simulink library "outp"  (R2021b)
settings: Solver=VariableStepAuto  StartTime=0.0  StopTime=10.0  RelTol=1e-3
undefined symbols (not defined in the file or in its folder): ENUM_PMMMODE_CHARGE, ENUM_PMMMODE_IDLE, ENUM_PMMMODE_INITIALIZE, ENUM_PMMMODE_POWERDOWN, ENUM_PMMMODE_SLEEP, Left, outp, slcm, TRUE
libraries: FVT_lib x686, hcu_lib x4, simulink x1
(part 4 of 7)

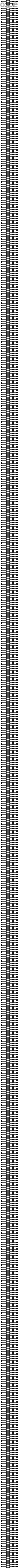
== system outp/OUTP/outpmodule ==
  VACC_HVTHCMSysAvail_enum : Inport
  VACC_LVBattVoltSta_enum : Inport  Port=2
  VACC_VehHVPwrAvail4THCM_W : Inport  Port=3
  VAPM_VehSpeed_kph : Inport  Port=4
  VAPM_VehSpeedTimeOut_flg : Inport  Port=5
  VAPM_FSOffSw_enum : Inport  Port=6
  VAPM_FSOffSwTimeOut_flg : Inport  Port=7
  VAPM_ChrgPlugSta_enum : Inport  Port=8
  VAPM_PASDRMR_cm : Inport  Port=9
  VAPM_PASDRML_cm : Inport  Port=10
  VAPM_PASDRCR_cm : Inport  Port=11
  VAPM_PASDRCL_cm : Inport  Port=12
  VAPM_PASDFMR_cm : Inport  Port=13
  VAPM_PASDFML_cm : Inport  Port=14
  VAPM_PASDFCR_cm : Inport  Port=15
  VAPM_PASDFCL_cm : Inport  Port=16
  VAPM_APSDRLR_cm : Inport  Port=17
  VAPM_APSDRLL_cm : Inport  Port=18
  VAPM_APSDFLR_cm : Inport  Port=19
  VAPM_APSDFLL_cm : Inport  Port=20
  VAPM_PASAFCL_enum : Inport  Port=21
  VAPM_PASARMR_enum : Inport  Port=22
  VAPM_PASARML_enum : Inport  Port=23
  VAPM_PASARCR_enum : Inport  Port=24
  VAPM_PASARCL_enum : Inport  Port=25
  VAPM_PASAFMR_enum : Inport  Port=26
  VAPM_PASAFML_enum : Inport  Port=27
  VAPM_PASAFCR_enum : Inport  Port=28
  VAPM_USSStaRMR_flg : Inport  Port=29
  VAPM_USSStaRML_flg : Inport  Port=30
  VAPM_USSStaRLR_flg : Inport  Port=31
  VAPM_USSStaRLL_flg : Inport  Port=32
  VAPM_USSStaRCR_flg : Inport  Port=33
  VAPM_USSStaRCL_flg : Inport  Port=34
  VAPM_USSStaFMR_flg : Inport  Port=35
  VAPM_USSStaFML_flg : Inport  Port=36
  VAPM_USSStaFLR_flg : Inport  Port=37
  VAPM_USSStaFLL_flg : Inport  Port=38
  VAPM_USSStaFCR_flg : Inport  Port=39
  VAPM_USSStaFCL_flg : Inport  Port=40
  VAPM_Chime_enum : Inport  Port=41
  VAPM_SNSRLayout_enum : Inport  Port=42
  VAPM_StaFSya_flg : Inport  Port=43
  VAPM_ModOperation_enum : Inport  Port=44
  VAPM_BrkPedalPos_pct : Inport  Port=45
  VAPM_BrkPedalPosTimeOut_flg : Inport  Port=46
  VAPM_LFRawWhlSpeed_kph : Inport  Port=47
  VAPM_LFRawWhlSpeedTimeOut_flg : Inport  Port=48
  VAPM_RFRawWhlSpeed_kph : Inport  Port=49
  VAPM_RFRawWhlSpeedTimeOut_flg : Inport  Port=50
  VAPM_LRRawWhlSpeed_kph : Inport  Port=51
  VAPM_LRRawWhlSpeedTimeOut_flg : Inport  Port=52
  VAPM_RRRawWhlSpeed_kph : Inport  Port=53
  VAPM_RRRawWhlSpeedTimeOut_flg : Inport  Port=54
  VAPM_LFRawWhlSpeedV_flg : Inport  Port=55
  VAPM_LFRawWhlSpeedVTimeOut_flg : Inport  Port=56
  VAPM_RFRawWhlSpeedV_flg : Inport  Port=57
  VAPM_RFRawWhlSpeedVTimeOut_flg : Inport  Port=58
  VAPM_LRRawWhlSpeedV_flg : Inport  Port=59
  VAPM_LRRawWhlSpeedVTimeOut_flg : Inport  Port=60
  VAPM_RRRawWhlSpeedV_flg : Inport  Port=61
  VAPM_RRRawWhlSpeedVTimeOut_flg : Inport  Port=62
  VAPM_LFWhlRotDir_enum : Inport  Port=63
  VAPM_LFWhlRotDirTimeOut_flg : Inport  Port=64
  VAPM_RFWhlRotDir_enum : Inport  Port=65
  VAPM_RFWhlRotDirTimeOut_flg : Inport  Port=66
  VAPM_LRWhlRotDir_enum : Inport  Port=67
  VAPM_LRWhlRotDirTimeOut_flg : Inport  Port=68
  VAPM_RRWhlRotDir_enum : Inport  Port=69
  VAPM_RRWhlRotDirTimeOut_flg : Inport  Port=70
  VAPM_LFPulseCountV_flg : Inport  Port=71
  VAPM_LFPulseCountVTimeOut_flg : Inport  Port=72
  VAPM_RFPulseCountV_flg : Inport  Port=73
  VAPM_RFPulseCountVTimeOut_flg : Inport  Port=74
  VAPM_LRPulseCountV_flg : Inport  Port=75
  VAPM_LRPulseCountVTimeOut_flg : Inport  Port=76
  VAPM_RRPulseCountV_flg : Inport  Port=77
  VAPM_RRPulseCountVTimeOut_flg : Inport  Port=78
  VAPM_LFPulseCount_enum : Inport  Port=79
  VAPM_LFPulseCountTimeOut_flg : Inport  Port=80
  VAPM_RFPulseCount_enum : Inport  Port=81
  VAPM_RFPulseCountTimeOut_flg : Inport  Port=82
  VAPM_LRPulseCount_enum : Inport  Port=83
  VAPM_LRPulseCountTimeOut_flg : Inport  Port=84
  VAPM_RRPulseCount_enum : Inport  Port=85
  VAPM_RRPulseCountTimeOut_flg : Inport  Port=86
  VAPM_ShifterHandleCmd_enum : Inport  Port=87
  VAPM_ShifterHandleCmdTimeOut_flg : Inport  Port=88
  VAPM_DriIntend_enum : Inport  Port=89
  VAPM_DriIntendTimeOut_flg : Inport  Port=90
  VAPM_EPSAOIControl_enum : Inport  Port=91
  VAPM_EPSAOIControlTimeOut_flg : Inport  Port=92
  VAPM_SASAngle_Deg : Inport  Port=93
  VAPM_SASAngleTimeOut_flg : Inport  Port=94
  VAPM_SASSpeed_degps : Inport  Port=95
  VAPM_SASSpeedTimeOut_flg : Inport  Port=96
  VAPM_SASSpeedValid_flg : Inport  Port=97
  VAPM_SASSpeedValidTimeOut_flg : Inport  Port=98
  VAPM_SASCAL_flg : Inport  Port=99
  VAPM_SASCALTimeOut_flg : Inport  Port=100
  VAPM_SASV_flg : Inport  Port=101
  VAPM_SASVTimeOut_flg : Inport  Port=102
  VAPM_GRADE_Deg : Inport  Port=103
  VAPM_GRADETimeOut_flg : Inport  Port=104
  VAPM_YawRate_degps : Inport  Port=105
  VAPM_YawRateTimeOut_flg : Inport  Port=106
  VAPM_LatAccel_Gps : Inport  Port=107
  VAPM_LatAccelTimeOut_flg : Inport  Port=108
  VAPM_LongAccel_Gps : Inport  Port=109
  VAPM_LongAccelTimeOut_flg : Inport  Port=110
  VAPM_MCPressure_bar : Inport  Port=111
  VAPM_MCPressureTimeOut_flg : Inport  Port=112
  VAPM_YawRateV_flg : Inport  Port=113
  VAPM_YawRateVTimeOut_flg : Inport  Port=114
  VAPM_LatAccelV_flg : Inport  Port=115
  VAPM_LatAccelVTimeOut_flg : Inport  Port=116
  VAPM_LongAccelV_flg : Inport  Port=117
  VAPM_LongAccelVTimeOut_flg : Inport  Port=118
  VAPM_MCPressureV_bar : Inport  Port=119
  VAPM_MCPressureVTimeOut_flg : Inport  Port=120
  VAPM_BrkSwSta_flg : Inport  Port=121
  VAPM_BrkSwStaTimeOut_flg : Inport  Port=122
  VAPM_BrkSwV_flg : Inport  Port=123
  VAPM_BrkSwVTimeOut_flg : Inport  Port=124
  VAPM_ESCStandstill_flg : Inport  Port=125
  VAPM_ESCStandstillTimeOut_flg : Inport  Port=126
  VAPM_ESCAPSSta_enum : Inport  Port=127
  VAPM_ESCAPSStaTimeOut_flg : Inport  Port=128
  VAPM_EPBExtReleaseAvail_flg : Inport  Port=129
  VAPM_EPBExtReleaseAvailTimeOut_flg : Inport  Port=130
  VAPM_EPBExtApplyAvail_flg : Inport  Port=131
  VAPM_EPBExtApplyAvailTimeOut_flg : Inport  Port=132
  VAPM_EPBErrSta_enum : Inport  Port=133
  VAPM_EPBErrStaTimeOut_flg : Inport  Port=134
  VAPM_EPBSta_enum : Inport  Port=135
  VAPM_EPBStaTimeOut_flg : Inport  Port=136
  VAPM_AVMparkingcancel_enum : Inport  Port=137
  VAPM_AVMparkingcancelTimeOut_flg : Inport  Port=138
  VAPM_AVMparkingexcute_enum : Inport  Port=139
  VAPM_AVMparkingexcuteTimeOut_flg : Inport  Port=140
  VAPM_AVMParkingmode_enum : Inport  Port=141
  VAPM_AVMParkingmodeTimeOut_flg : Inport  Port=142
  VAPM_AVMErrSTA_flg : Inport  Port=143
  VAPM_AVMErrSTATimeOut_flg : Inport  Port=144
  VAPM_IVIStatus_flg : Inport  Port=145
  VAPM_IVIStatusTimeOut_flg : Inport  Port=146
  VAPM_CAASSw_enum : Inport  Port=147
  VAPM_CAASSwTimeOut_flg : Inport  Port=148
  VAPM_IVIScreen_enum : Inport  Port=149
  VAPM_IVIScreenTimeOut_flg : Inport  Port=150
  VAPM_ABSActive_flg : Inport  Port=151
  VAPM_ABSActiveTimeOut_flg : Inport  Port=152
  VAPM_TCSActive_flg : Inport  Port=153
  VAPM_TCSActiveTimeOut_flg : Inport  Port=154
  VAPM_DriverSeatBeltCmd_flg : Inport  Port=155
  VAPM_DriverSeatBeltCmdTimeOut_flg : Inport  Port=156
  VAPM_APSProgressPCT_pct : Inport  Port=157
  VAPM_APSRQDisplay_enum : Inport  Port=158
  VAPM_APSSWVer_enum : Inport  Port=159
  VAPM_APSHWVer_enum : Inport  Port=160
  VAPM_APSExitCondition_enum : Inport  Port=161
  VAPM_APSAngleTarget_Deg : Inport  Port=162
  VAPM_APSVRqEPASCtrl_flg : Inport  Port=163
  VAPM_APSRqEPASCtrl_flg : Inport  Port=164
  VAPM_CAASSta_enum : Inport  Port=165
  VBCM_AntitheftSta_enum : Inport  Port=166
  VBCM_TailgateRemote_enum : Inport  Port=167
  VBCM_HornCtrl_flg : Inport  Port=168
  VBCM_AllDoorSW_flg : Inport  Port=169
  VBCM_BCMDoorLockSta_flg : Inport  Port=170
  VBCM_AntitheftSeatFlod_flg : Inport  Port=171
  VBCM_HoodSW_flg : Inport  Port=172
  VBCM_TailgateSW_flg : Inport  Port=173
  VBCM_DrDoorSW_flg : Inport  Port=174
  VBCM_PsDoorSW_flg : Inport  Port=175
  VBCM_RLDoorSW_flg : Inport  Port=176
  VBCM_RRDoorSW_flg : Inport  Port=177
  VBCM_LockSetting_flg : Inport  Port=178
  VBCM_FrChargingDoorCtrl_enum : Inport  Port=179
  VBCM_RrChargingDoorCtrl_enum : Inport  Port=180
  VBCM_CrashDetd_flg : Inport  Port=181
  VBCM_CTDCtrl_enum : Inport  Port=182
  VBCM_DoorLockIND_flg : Inport  Port=183
  VBCM_CTDLockSW_flg : Inport  Port=184
  VBCM_Dimmer_pct : Inport  Port=185
  VBCM_DimmerEN_flg : Inport  Port=186
  VBCM_PosLamp_flg : Inport  Port=187
  VBCM_LBeam_flg : Inport  Port=188
  VBCM_HBeam_flg : Inport  Port=189
  VBCM_RrFogLamp_flg : Inport  Port=190
  VBCM_BrakeLamp_flg : Inport  Port=191
  VBCM_ReverseLamp_flg : Inport  Port=192
  VBCM_LDRL_flg : Inport  Port=193
  VBCM_RDRL_flg : Inport  Port=194
  VBCM_LBSD_flg : Inport  Port=195
  VBCM_RBSD_flg : Inport  Port=196
  VBCM_HazardSW_flg : Inport  Port=197
  VBCM_LTurnLP_flg : Inport  Port=198
  VBCM_RTurnLP_flg : Inport  Port=199
  VBCM_BCMBuzzerReq_flg : Inport  Port=200
  VBCM_MirrorCtrl_enum : Inport  Port=201
  VBCM_MirrorDefog_flg : Inport  Port=202
  VBCM_RrDefog_flg : Inport  Port=203
  VBCM_RoomLampH_flg : Inport  Port=204
  VBCM_RoomLampL_flg : Inport  Port=205
  VBCM_TrunkRel_flg : Inport  Port=206
  VBCM_TailgateHDSW_flg : Inport  Port=207
  VBCM_FrWiperL_flg : Inport  Port=208
  VBCM_FrWiperH_flg : Inport  Port=209
  VBCM_RrWiper_flg : Inport  Port=210
  VBCM_WasherCtrl_enum : Inport  Port=211
  VBCM_WiperFixMode_flg : Inport  Port=212
  VBCM_AmbLightBreath1_enum : Inport  Port=213
  VBCM_AmbLightBreath2_enum : Inport  Port=214
  VBCM_AmbLightBreath3_enum : Inport  Port=215
  VBCM_AmbLightBreath4_enum : Inport  Port=216
  VBCM_AmbLightBreath5_enum : Inport  Port=217
  VBCM_AmbLightBreath6_enum : Inport  Port=218
  VBCM_AmbLightBrightness1_enum : Inport  Port=219
  VBCM_AmbLightBrightness2_enum : Inport  Port=220
  VBCM_AmbLightBrightness3_enum : Inport  Port=221
  VBCM_AmbLightBrightness4_enum : Inport  Port=222
  VBCM_AmbLightBrightness5_enum : Inport  Port=223
  VBCM_AmbLightBrightness6_enum : Inport  Port=224
  VBCM_AmbLightColor1_enum : Inport  Port=225
  VBCM_AmbLightColor2_enum : Inport  Port=226
  VBCM_AmbLightColor3_enum : Inport  Port=227
  VBCM_AmbLightColor4_enum : Inport  Port=228
  VBCM_AmbLightColor5_enum : Inport  Port=229
  VBCM_AmbLightColor6_enum : Inport  Port=230
  VBCM_LampPwr_flg : Inport  Port=231
  VBCM_SPTGDet_flg : Inport  Port=232
  VBCM_APSOpenPTG_flg : Inport  Port=233
  VBCM_FollowMe_flg : Inport  Port=234
  VBCM_IVIRST_flg : Inport  Port=235
  VBCM_CountAlarm_enum : Inport  Port=236
  VBCM_MFSWTri_flg : Inport  Port=237
  VBCM_MirrorFlodPos_flg : Inport  Port=238
  VBCM_FuelDoorPos_flg : Inport  Port=239
  VBCM_MFRDNBrightReq_pct : Inport  Port=240
  VBCM_RoomLampMode_flg : Inport  Port=241
  VBCM_IVIPTGUSStaSW_flg : Inport  Port=242
  VBCM_PTGInnerSW2_enum : Inport  Port=243
  VBCM_LDrvCtrlCmd_pct : Inport  Port=244
  VBCM_LPasCtrlCmd_pct : Inport  Port=245
  VBCM_LRLDCtrlCmd_pct : Inport  Port=246
  VBCM_LRRDCtrlCmd_pct : Inport  Port=247
  VBCM_APMDoorControlSta_flg : Inport  Port=248
  VBCM_AmbFunEN_flg : Inport  Port=249
  VBCM_AmbWelEN_flg : Inport  Port=250
  VBCM_AmbDimEN_flg : Inport  Port=251
  VBCM_AmbLinkDriSta_flg : Inport  Port=252
  VBCM_AmbPwrWarnEN_flg : Inport  Port=253
  VBCM_AmbODAEN_flg : Inport  Port=254
  VBCM_AmbColorSta_enum : Inport  Port=255
  VBCM_AmbBrightSta_enum : Inport  Port=256
  VBCM_LockAlarm_enum : Inport  Port=257
  VBCM_ATCtrl_enum : Inport  Port=258
  VBCM_fUnlockSingle_flg : Inport  Port=259
  VBCM_UserNow_enum : Inport  Port=260
  VBCM_AmbFunENFlash_enum : Inport  Port=261
  VBCM_AmbWelENFlash_enum : Inport  Port=262
  VBCM_AmbDimENFlash_enum : Inport  Port=263
  VBCM_AmbLinkDriStaFlash_enum : Inport  Port=264
  VBCM_AmbPwrWarnENFlash_enum : Inport  Port=265
  VBCM_AmbODAENFlash_enum : Inport  Port=266
  VBCM_AmbColorSta1_enum : Inport  Port=267
  VBCM_AmbColorSta2_enum : Inport  Port=268
  VBCM_AmbColorSta3_enum : Inport  Port=269
  VBCM_AmbColorSta4_enum : Inport  Port=270
  VBCM_AmbColorSta5_enum : Inport  Port=271
  VBCM_AmbColorSta7_enum : Inport  Port=272
  VBCM_AmbBrightnessSta1_enum : Inport  Port=273
  VBCM_AmbBrightnessSta2_enum : Inport  Port=274
  VBCM_AmbBrightnessSta3_enum : Inport  Port=275
  VBCM_AmbBrightnessSta4_enum : Inport  Port=276
  VBCM_AmbBrightnessSta5_enum : Inport  Port=277
  VBCM_AmbBrightnessSta7_enum : Inport  Port=278
  VBCM_HazardIND_flg : Inport  Port=279
  VBCM_DimSwSta_flg : Inport  Port=280
  VBCM_PassSWSta_flg : Inport  Port=281
  VBCM_FWipSwSta_enum : Inport  Port=282
  VBCM_FWasSwSta_enum : Inport  Port=283
  VBCM_TurnSwSta_enum : Inport  Port=284
  VDHP_ActAPSPosn_pct : Inport  Port=285
  VDHP_EAPS1MIN_pct : Inport  Port=286
  VDHP_EAPS2MIN_pct : Inport  Port=287
  VDKC_DKCTimeSN_cnt : Inport  Port=288
  VDKC_DKCAuthSta_enum : Inport  Port=289
  VDSC_DISCTurn_flg : Inport  Port=290
  VDSC_DISCTargetSpd_kph : Inport  Port=291
  VDSC_DISCSta_enum : Inport  Port=292
  VDSC_DISCButtSta_flg : Inport  Port=293
  VNMM_AllCANTxReq_flg : Inport  Port=294
  VNMM_NMmTxReq_flg : Inport  Port=295
  VNMM_Awake_enum : Inport  Port=296
  VNMM_CSB_flg : Inport  Port=297
  VNMM_ErrorState_enum : Inport  Port=298
  VNMM_NodeID_enum : Inport  Port=299
  VNMM_PNI_flg : Inport  Port=300
  VNMM_RptMsgReq_flg : Inport  Port=301
  VNMM_WakeUp_enum : Inport  Port=302
  VNMM_ActiveWU_flg : Inport  Port=303
  VNMM_SysNMmSta_enum : Inport  Port=304
  VNMM_NetworkReq_flg : Inport  Port=305
  VPMM_PowerUpState_enum : Inport  Port=306
  VPMM_PowerDownState_enum : Inport  Port=307
  VPMM_PowerUpFault_enum : Inport  Port=308
  VPMM_PowerDownFault_enum : Inport  Port=309
  VPMM_ActiveDischargeReq_flg : Inport  Port=310
  VPMM_DCDCEnaReq_flg : Inport  Port=311
  VPMM_DCDCVoltSetpoint_V : Inport  Port=312
  VPMM_HVBatCnctReq_flg : Inport  Port=313
  VPMM_HVSysReadyToCharge_enum : Inport  Port=314
  VPMM_PowerSta_enum : Inport  Port=315
  VPMM_LVPwrSta_flg : Inport  Port=316
  VPMM_HVPwrSta_flg : Inport  Port=317
  VPMM_SysPowerMode_enum : Inport  Port=318
  VPMM_FrMCUEnaReq_flg : Inport  Port=319
  VPMM_RrMCUEnaReq_flg : Inport  Port=320
  VPMM_DrivetrainSelect_enum : Inport  Port=321
  VPMM_DrSeatSta_enum : Inport  Port=322
  VPMM_PwrStaSelect_enum : Inport  Port=323
  VPMM_PwrStaConstraint_enum : Inport  Port=324
  VPMM_TCountSta_enum : Inport  Port=325
  VPMM_PwrUpReq_enum : Inport  Port=326
  VPMM_PwrDownReq_enum : Inport  Port=327
  VPMM_LowSOCWarn_enum : Inport  Port=328
  VPMM_ReVehThdChkSta_enum : Inport  Port=329
  VPMM_LVSysErrPwrOutErr_flg : Inport  Port=330
  VPMM_EvccAplusPwrUpReq_flg : Inport  Port=331
  VPMM_PwrStaONTOPopReq_flg : Inport  Port=332
  VPMM_IVIPwrStaONTOPopT_s : Inport  Port=333
  VPMM_LVChrgHoldTtimer_s : Inport  Port=334
  VPMM_LVBattChrgTimeCnt_s : Inport  Port=335
  VPMM_SilentChkAllowSleep_flg : Inport  Port=336
  VPMM_TimerAllowSleep_flg : Inport  Port=337
  VPMM_FDADC12VDetAvg_mV : Inport  Port=338
  VPMM_PMMAllowECUSleep_flg : Inport  Port=339
  VPMM_LVSilentChrgSta_enum : Inport  Port=340
  VPMM_LVSilentChrgReq_flg : Inport  Port=341
  VPMM_LVSilentChrgLv_enum : Inport  Port=342
  VPMM_CtrlFrPwrStbA1P_flg : Inport  Port=343
  VPMM_CtrlFrRC1_flg : Inport  Port=344
  VPMM_CtrlFrBMSCCUCIR_flg : Inport  Port=345
  VPMM_CtrlFrEDUINVERTER_flg : Inport  Port=346
  VPMM_HWResetSta_enum : Inport  Port=347
  VPMM_CtrlDrPwrStbA2_flg : Inport  Port=348
  VPMM_PwrStaTOSta_enum : Inport  Port=349
  VPMM_Sched_ChgTOSta_enum : Inport  Port=350
  VPMM_PwrReq_OTA_enum : Inport  Port=351
  VPMM_OTAPwrReqOFFChkSta_enum : Inport  Port=352
  VPMM_OTAPwrReqStdChkSta_enum : Inport  Port=353
  VSYS_HWVer1_cnt : Inport  Port=354
  VSYS_HWVer2_cnt : Inport  Port=355
  VSYS_HWVer3_cnt : Inport  Port=356
  VSYS_CarModel1_cnt : Inport  Port=357
  VSYS_CarModel2_cnt : Inport  Port=358
  VSYS_CarModel3_cnt : Inport  Port=359
  VSYS_ECU1_cnt : Inport  Port=360
  VSYS_ECU2_cnt : Inport  Port=361
  VSYS_Major1_cnt : Inport  Port=362
  VSYS_Major2_cnt : Inport  Port=363
  VSYS_Minor1_cnt : Inport  Port=364
  VSYS_Minor2_cnt : Inport  Port=365
  VSYS_Patch1_cnt : Inport  Port=366
  VSYS_Patch2_cnt : Inport  Port=367
  VSYS_Country1_cnt : Inport  Port=368
  VSYS_Country2_cnt : Inport  Port=369
  VSYS_Variation_cnt : Inport  Port=370
  VSYS_Dash1_cnt : Inport  Port=371
  VSYS_Change1_cnt : Inport  Port=372
  VSYS_Change2_cnt : Inport  Port=373
  VSYS_Dash2_cnt : Inport  Port=374
  VSYS_SHA1_cnt : Inport  Port=375
  VSYS_SHA2_cnt : Inport  Port=376
  VSYS_SHA3_cnt : Inport  Port=377
  VSYS_SHA4_cnt : Inport  Port=378
  VSYS_SHA5_cnt : Inport  Port=379
  VSYS_SHA6_cnt : Inport  Port=380
  VSYS_SHA7_cnt : Inport  Port=381
  VSYS_SHA8_cnt : Inport  Port=382
  VSYS_NvWriteReqRisingEdge_flg : Inport  Port=383
  VSYS_FdcSlpReqRisingEdge_flg : Inport  Port=384
  VSYS_FdcSlpTime_sec : Inport  Port=385
  VSYS_PmicBootReason_enum : Inport  Port=386
  VSYS_WisrBootReason_raw32 : Inport  Port=387
  VSYS_AcoreRebootCmdACK_flg : Inport  Port=388
  VSYS_CurrentNmState_enum : Inport  Port=389
  VTHC_FDCompCmd_rpm : Inport  Port=390
  VTHC_FDSOV1Cmd_flg : Inport  Port=391
  VTHC_FDSOV2Cmd_flg : Inport  Port=392
  VTHC_FDSOV3Cmd_flg : Inport  Port=393
  VTHC_FDEXV1Cmd_step : Inport  Port=394
  VTHC_FDEXV2Cmd_step : Inport  Port=395
  VTHC_FDSOTXVCmd_flg : Inport  Port=396
  VTHC_FDFWVCmd_flg : Inport  Port=397
  VTHC_FDTWVCmd_pct : Inport  Port=398
  VTHC_FDFrWPTCHeatPwrCmd_W : Inport  Port=399
  VTHC_CoolgFanActDuty_pct : Inport  Port=400
  VTHC_FDAGSCmd_enum : Inport  Port=401
  VTHC_FDEWP1Cmd_enum : Inport  Port=402
  VTHC_FDEWP2Cmd_enum : Inport  Port=403
  VTHC_FDEWP3Cmd_enum : Inport  Port=404
  VTHC_FDFrLeAPTCHeatPwrCmd_W : Inport  Port=405
  VTHC_FDFrRiAPTCHeatPwrCmd_W : Inport  Port=406
  VTHC_FDRrAPTCHeatPwrCmd_W : Inport  Port=407
  VTHC_FDBlowerCmd_pct : Inport  Port=408
  VTHC_BatteryMode_enum : Inport  Port=409
  VTHC_EDriveMode_enum : Inport  Port=410
  VTHC_CabinMode_enum : Inport  Port=411
  VTHC_CCUACLampSts_flg : Inport  Port=412
  VTHC_CCUAutoLampSts_flg : Inport  Port=413
  VTHC_CCUACMaxLampSts_flg : Inport  Port=414
  VTHC_CCUSyncLampSts_flg : Inport  Port=415
  VTHC_sigAirIntenZon1St_enum : Inport  Port=416
  VTHC_sigWindDirZon1St_enum : Inport  Port=417
  VTHC_sigRecircSt_flg : Inport  Port=418
  VTHC_sigSetTempZon1St_C : Inport  Port=419
  VTHC_sigSetTempZon2St_C : Inport  Port=420
  VTHC_sigClntTHvBattOut_C : Inport  Port=421
  VTHC_sigCbnSolarLeft_W : Inport  Port=422
  VTHC_sigClntTHvBattIn_C : Inport  Port=423
  VTHC_sigCbnSolarRight_W : Inport  Port=424
  VTHC_sigAmbAirT_C : Inport  Port=425
  VTHC_sigCbnAirT_C : Inport  Port=426
  VTHC_ACSubMode_enum : Inport  Port=427
  VTHC_FDRecyAutoCmd_enum : Inport  Port=428
  VTHC_ACModeMem_enum : Inport  Port=429
  VTHC_Face_flg : Inport  Port=430
  VTHC_Foot_flg : Inport  Port=431
  VTHC_Frost_flg : Inport  Port=432
  VTHC_FaceM_flg : Inport  Port=433
  VTHC_FootM_flg : Inport  Port=434
  VTHC_CCUSyncSts_flg : Inport  Port=435
  VTHC_ACForceOFF_flg : Inport  Port=436
  VTHC_RecAutoFlg_flg : Inport  Port=437
  VTHC_AirIntenZone1M_enum : Inport  Port=438
  VTHC_fdefog_flg : Inport  Port=439
  VTHC_sigSetTempZon2StM_C : Inport  Port=440
  VTHC_FDCTHCMAPTCWarningSta_flg : Inport  Port=441
  VTPM_LFBatWarn_flg : Inport  Port=442
  VTPM_RFBatWarn_flg : Inport  Port=443
  VTPM_LRBatWarn_flg : Inport  Port=444
  VTPM_RRBatWarn_flg : Inport  Port=445
  VTPM_LFWheelPress_raw8 : Inport  Port=446
  VTPM_RFWheelPress_raw8 : Inport  Port=447
  VTPM_LRWheelPress_raw8 : Inport  Port=448
  VTPM_RRWheelPress_raw8 : Inport  Port=449
  VTPM_LFWheelTemp_C : Inport  Port=450
  VTPM_RFWheelTemp_C : Inport  Port=451
  VTPM_LRWheelTemp_C : Inport  Port=452
  VTPM_RRWheelTemp_C : Inport  Port=453
  VTPM_LFSensorFail_flg : Inport  Port=454
  VTPM_RFSensorFail_flg : Inport  Port=455
  VTPM_LRSensorFail_flg : Inport  Port=456
  VTPM_RRSensorFail_flg : Inport  Port=457
  VTPM_LFWheelDebug_flg : Inport  Port=458
  VTPM_LRWheelDebug_flg : Inport  Port=459
  VTPM_RFWheelDebug_flg : Inport  Port=460
  VTPM_RRWheelDebug_flg : Inport  Port=461
  VTPM_TPMSResButtAllow_flg : Inport  Port=462
  VTPM_TPMSCaliButtAllow_flg : Inport  Port=463
  VTPM_LFPressIndi_enum : Inport  Port=464
  VTPM_RFPressIndi_enum : Inport  Port=465
  VTPM_LRPressIndi_enum : Inport  Port=466
  VTPM_RRPressIndi_enum : Inport  Port=467
  VTPM_TPMSWarnIndi_enum : Inport  Port=468
  VTPM_LFWheelTmpIndi_flg : Inport  Port=469
  VTPM_RFWheelTmpIndi_flg : Inport  Port=470
  VTPM_LRWheelTmpIndi_flg : Inport  Port=471
  VTPM_RRWheelTmpIndi_flg : Inport  Port=472
  VTPM_LFWheelPSW_raw8 : Inport  Port=473
  VTPM_LRWheelPSW_raw8 : Inport  Port=474
  VTPM_RFWheelPSW_raw8 : Inport  Port=475
  VTPM_RRWheelPSW_raw8 : Inport  Port=476
  VTPM_CWheelTips_enum : Inport  Port=477
  VTPM_AutoLTips_enum : Inport  Port=478
  VTPM_LFSensorMode_flg : Inport  Port=479
  VTPM_RFSensorMode_flg : Inport  Port=480
  VTPM_LRSensorMode_flg : Inport  Port=481
  VTPM_RRSensorMode_flg : Inport  Port=482
  VTPM_S1ID_raw32 : Inport  Port=483
  VTPM_S2ID_raw32 : Inport  Port=484
  VTPM_S3ID_raw32 : Inport  Port=485
  VTPM_S4ID_raw32 : Inport  Port=486
  VTPM_S1L_enum : Inport  Port=487
  VTPM_S2L_enum : Inport  Port=488
  VTPM_S3L_enum : Inport  Port=489
  VTPM_S4L_enum : Inport  Port=490
  VTPM_ALFin_flg : Inport  Port=491
  VTPM_LFP20_raw8 : Inport  Port=492
  VTPM_RFP20_raw8 : Inport  Port=493
  VTPM_LRP20_raw8 : Inport  Port=494
  VTPM_RRP20_raw8 : Inport  Port=495
  VTPM_FAT_flg : Inport  Port=496
  VTPM_IDin_raw32 : Inport  Port=497
  VTPM_S1WheelDebugALTU_pct : Inport  Port=498
  VTPM_S2WheelDebugALTU_pct : Inport  Port=499
  VTPM_S3WheelDebugALTU_pct : Inport  Port=500
  VTPM_S4WheelDebugALTU_pct : Inport  Port=501
  VTPM_ID1messageALTU_raw8 : Inport  Port=502
  VTPM_ID2messageALTU_raw8 : Inport  Port=503
  VTPM_ID3messageALTU_raw8 : Inport  Port=504
  VTPM_ID4messageALTU_raw8 : Inport  Port=505
  VTPM_Chkfin_flg : Inport  Port=506
  VTPM_SetIDLoc_flg : Inport  Port=507
  VTPM_TPMSStorge_flg : Inport  Port=508
  VTPM_ChkStorge_flg : Inport  Port=509
  VTPM_TPMSResButt_flg : Inport  Port=510
  VTPM_LFPindi_enum : Inport  Port=511
  VTPM_RFPind_enum : Inport  Port=512
  VTPM_LRPindi_enum : Inport  Port=513
  VTPM_RRPindi_enum : Inport  Port=514
  VTPM_WriteChkLFID_raw : Inport  Port=515
  VTPM_WriteChkRFID_raw : Inport  Port=516
  VTPM_WriteChkLRID_raw : Inport  Port=517
  VTPM_WriteChkRRID_raw : Inport  Port=518
  VTPM_WriteChkfinLFID_raw : Inport  Port=519
  VTPM_WriteChkfinRFID_raw : Inport  Port=520
  VTPM_WriteChkfinLRID_raw : Inport  Port=521
  VTPM_WriteChkfinRRID_raw : Inport  Port=522
  VTPM_Flashchkdatavalid_enum : Inport  Port=523
  VTPM_Flashdatavalid_enum : Inport  Port=524
  VTPM_unlearnSfali_flg : Inport  Port=525
  VTPM_unlearnSfailvalid_enum : Inport  Port=526
  VTPM_Prepresstempvalid_enum : Inport  Port=527
  VTPM_FlashS1ID_raw : Inport  Port=528
  VTPM_FlashS2ID_raw : Inport  Port=529
  VTPM_FlashS3ID_raw : Inport  Port=530
  VTPM_FlashS4ID_raw : Inport  Port=531
  VTPM_FlashIDvalid_enum : Inport  Port=532
  VTQD_ParkRequest_flg : Inport  Port=533
  VTQD_TqSourceFr_enum : Inport  Port=534
  VTQD_TqSourceRr_enum : Inport  Port=535
  VTQD_FrEDUAvailBrkRgnTq_Nm : Inport  Port=536
  VTQD_RrEDUAvailBrkRgnTq_Nm : Inport  Port=537
  VTQD_EVDriveMode_enum : Inport  Port=538
  VTQD_ShiftGearPosn_enum : Inport  Port=539
  VTQD_PButtonSta_enum : Inport  Port=540
  VTQD_FrActvDmpDisabReq_flg : Inport  Port=541
  VTQD_RrActvDmpDisabReq_flg : Inport  Port=542
  VTQD_FrRgnDecrSta_flg : Inport  Port=543
  VTQD_RrRgnDecrSta_flg : Inport  Port=544
  VTQD_DriverWhlTqDemFr_Nm : Inport  Port=545
  VTQD_DriverWhlTqDemRr_Nm : Inport  Port=546
  VTQD_FrEDUActTq_Nm : Inport  Port=547
  VTQD_RrEDUActTq_Nm : Inport  Port=548
  VTQD_FrEDURolRgnTq_Nm : Inport  Port=549
  VTQD_RrEDURolRgnTq_Nm : Inport  Port=550
  VTQD_FrEDUSpd_rpm : Inport  Port=551
  VTQD_RrEDUSpd_rpm : Inport  Port=552
  VTQD_FrEDUSpdValid_flg : Inport  Port=553
  VTQD_FrEDUAvailBrkRgnTqV_flg : Inport  Port=554
  VTQD_RrEDUSpdValid_flg : Inport  Port=555
  VTQD_RrEDUAvailBrkRgnTqV_flg : Inport  Port=556
  VTQD_RgnAbnorSta_flg : Inport  Port=557
  VTQD_PTCSPermSta_flg : Inport  Port=558
  VTQD_FrRgnPermSta_flg : Inport  Port=559
  VTQD_RrRgnPermSta_flg : Inport  Port=560
  VTQD_FrIdcMin_A : Inport  Port=561
  VTQD_FrIdcMax_A : Inport  Port=562
  VTQD_FrUdcMin_V : Inport  Port=563
  VTQD_FrUdcMax_V : Inport  Port=564
  VTQD_RrIdcMin_A : Inport  Port=565
  VTQD_RrIdcMax_A : Inport  Port=566
  VTQD_RrUdcMin_V : Inport  Port=567
  VTQD_RrUdcMax_V : Inport  Port=568
  VTQD_ReBrakeLPReq_flg : Inport  Port=569
  VTQD_CreepON_flg : Inport  Port=570
  VTQD_EquivAccPedalSWSta_flg : Inport  Port=571
  VTQD_DriveProtEn_flg : Inport  Port=572
  VTQD_ActParkRequest_flg : Inport  Port=573
  VTQD_IVIPwrLockSta_enum : Inport  Port=574
  VTQD_OPDHoldLamp_flg : Inport  Port=575
  VTQD_SaveRegenMode_enum : Inport  Port=576
  VTQD_FDCVCURegenMode_enum : Inport  Port=577
  VTQD_SpdCtrlMode_enum : Inport  Port=578
  VTQD_SpdCtrlSta_flg : Inport  Port=579
  VTQD_SetSpd_kph : Inport  Port=580
  VTQR_FrTMTqReq_Nm : Inport  Port=581
  VTQR_RrTMTqReq_Nm : Inport  Port=582
  VV2L_ReqOBCV2LEna_enum : Inport  Port=583
  VV2L_ReqV2LIVIPopup_enum : Inport  Port=584
  VVMC_FeatSetSpdFinal_raw32 : Inport  Port=585
  VVMC_VehicleSpeed_mph : Inport  Port=586
  VVMC_VehicleSpeed_kph : Inport  Port=587
  VVMC_MeterIndSpeed_raw32 : Inport  Port=588
  VVMC_VMCAEBCtrlAvail_flg : Inport  Port=589
  VVMC_VMCACCCtrlAvail_flg : Inport  Port=590
  VVMC_VMCCCCtrlAvail_flg : Inport  Port=591
  VVMC_VMCMSACtrlAvail_flg : Inport  Port=592
  VVMC_FeatArbitrSta_enum : Inport  Port=593
  VVMC_FeatReqSpd_kph : Inport  Port=594
  VVMC_JerkPCT_pct : Inport  Port=595
  VVMC_LimitPCT_pct : Inport  Port=596
  VVMC_FrontRearSlipRatioCtrl_flg : Inport  Port=597
  VVMC_RearWhlSlipRatioCtrl_flg : Inport  Port=598
  VVMC_SingleWhlSlipRatioCtrl_flg : Inport  Port=599
  VVMC_LatAccCtrl_flg : Inport  Port=600
  VVMC_SafetyCtrl_flg : Inport  Port=601
  VVMC_SPD2ACCAct_flg : Inport  Port=602
  VVMC_AccCalcuPID_mps2 : Inport  Port=603
  VVMC_ISOAccLimit_mps2 : Inport  Port=604
  VVMC_ISODecLimit_mps2 : Inport  Port=605
  VVMC_ISOJerkLimit_mps3 : Inport  Port=606
  VVMC_ACCRequiredAccel_mps2 : Inport  Port=607
  VVMC_DISCReqAcc_mps2 : Inport  Port=608
  VVMC_FeatArbitrFinal_enum : Inport  Port=609
  VVMC_LateralCtrl_flg : Inport  Port=610
  VVMC_ADASLKASta_enum : Inport  Port=611
  VVMC_LKAStrToqReq_Nm : Inport  Port=612
  VVMC_LKATOIFault_flg : Inport  Port=613
  VVMC_LKATOIAct_enum : Inport  Port=614
  VVMC_ADASAEBReq_enum : Inport  Port=615
  VVMC_ADASFaultSta_flg : Inport  Port=616
  VVMC_AEBVehHoldReq_flg : Inport  Port=617
  VVMC_ACCVehHoldReq_flg : Inport  Port=618
  VVMC_ADASDBSReq_enum : Inport  Port=619
  VVMC_ADASACCSta_enum : Inport  Port=620
  VVMC_ACCObjDist_m : Inport  Port=621
  VVMC_ACCObjRelSpd_mps : Inport  Port=622
  VVMC_TimeGapLevel_enum : Inport  Port=623
  VVMC_ACCJerkUpperLimit_mps3 : Inport  Port=624
  VVMC_ACCComfortBandUpper_mps2 : Inport  Port=625
  VVMC_ACCJerkLowerLimit_mps3 : Inport  Port=626
  VVMC_ACCComfortBandLower_mps2 : Inport  Port=627
  VVMC_ADASVehSpdLim_raw32 : Inport  Port=628
  VVMC_ADASShftPosnReqA_flg : Inport  Port=629
  VVMC_ADASShftPosnReq_enum : Inport  Port=630
  VVMC_ADASForceIdle_flg : Inport  Port=631
  VVMC_HazardWarningReq_flg : Inport  Port=632
  VVMC_RightTurnLightReq_flg : Inport  Port=633
  VVMC_LeftTurnLightReq_flg : Inport  Port=634
  VVMC_ADASFCWSta_enum : Inport  Port=635
  VVMC_ADASLDWSta_enum : Inport  Port=636
  VVMC_ADASFltWrnReq_flg : Inport  Port=637
  VVMC_ACCObjDstLvl_enum : Inport  Port=638
  VVMC_ForceLowBeam_enum : Inport  Port=639
  VVMC_ACCTakeoverReq_flg : Inport  Port=640
  VVMC_ADASWarningMsg_enum : Inport  Port=641
  VVMC_ADASCAMSpdLim_enum : Inport  Port=642
  VVMC_TargetType_enum : Inport  Port=643
  VVMC_ADASSLIFSpdLim_enum : Inport  Port=644
  VVMC_LKAHODDisplayWarning_flg : Inport  Port=645
  VVMC_LKAHODSoundWarning_flg : Inport  Port=646
  VVMC_ADASLFCSta_enum : Inport  Port=647
  VVMC_ADASLaneModeL_enum : Inport  Port=648
  VVMC_ADASLaneModeR_enum : Inport  Port=649
  VVMC_ADASSLIFSta_enum : Inport  Port=650
  VVMC_ADASISASta_enum : Inport  Port=651
  VVMC_ADASLDWMute_flg : Inport  Port=652
  VVMC_ADASFCWMute_flg : Inport  Port=653
  VVMC_ADASLFCHandsOffWarning_enum : Inport  Port=654
  VVMC_LVDADisabled_flg : Inport  Port=655
  VVMC_LVDAMuteSta_enum : Inport  Port=656
  VVMC_LVDAFailinfo_flg : Inport  Port=657
  VVMC_LVDAWarning_flg : Inport  Port=658
  VVMC_LVDAACCStatusInformation_flg : Inport  Port=659
  VVMC_ADASLFCWarnSound_enum : Inport  Port=660
  VVMC_FCMACCmode_enum : Inport  Port=661
  VVMC_ADASLanetypeR_enum : Inport  Port=662
  VVMC_ADASLanetypeL_enum : Inport  Port=663
  VVMC_ADASLanecurveL_raw32 : Inport  Port=664
  VVMC_ADASLanecurveR_raw32 : Inport  Port=665
  VVMC_ADASAEBSta_enum : Inport  Port=666
  VVMC_FCMLDWRequest_enum : Inport  Port=667
  VVMC_FCMLDWFault_flg : Inport  Port=668
  VVMC_ACCCtrlAvail_flg : Inport  Port=669
  VVMC_ACCPedalOvrd_flg : Inport  Port=670
  VVMC_TimeGapCalcu_s : Inport  Port=671
  VVMC_CCCtrlSta_enum : Inport  Port=672
  VVMC_MSACtrlSta_enum : Inport  Port=673
  VVMC_APSCtrlAvail_flg : Inport  Port=674
  VVMC_APSStaSys_enum : Inport  Port=675
  VVMC_APSDecReqA_flg : Inport  Port=676
  VVMC_APSDecReq_mps2 : Inport  Port=677
  VVMC_APSReq_enum : Inport  Port=678
  VVMC_CCMSASpdWar_flg : Inport  Port=679
  VVMC_IMUEnaCmd_flg : Inport  Port=680
  VVMC_CAASCtrlAvail_flg : Inport  Port=681
  VVMC_CAASActive_flg : Inport  Port=682
  VVMC_VMCRWSActvSta_enum : Inport  Port=683
  VVMC_VMCRWSDfctvSta_enum : Inport  Port=684
  VVMC_VMCRWSPositionReq_mm : Inport  Port=685
  VVMC_VMCSteerFaultRequest_enum : Inport  Port=686
  UnitConverter{1..2,6,8..16,21..28,41..42,44,63,65,67,69,79,81,83,85,87,89,91,127,133,135,137,139,141,147,149,158..161,165..167,179..180,182,201,211,213..230,236,240,243..247,255..258,260..278,282..284,289,292,296,298..299,302,304,306..309,314..315,318,321..329,340,342,347,349..382,386,389,401..404,409..411,416..417,427..429,438,446..449,464..468,473..478,487..490,492..495,502..505,511..514,523..524,526..527,532,534..535,538..540,574,576..578,583..584,593,609,611,614..615,619..620,623,630,635..636,638..639,641..644,647..651,654,656,660..663,666..667,672..673,675,678,683..684,686} (264 alike) : DataTypeConversion  OutDataTypeStr=uint8
  UnitConverter{5,7,29..40,43,46,48,50,52,54..62,64,66,68,70..78,80,82,84,86,88,90,92,94,96..102,104,106,108,110,112..126,128..132,134,136,138,140,142..146,148,150..156,163..164,168..178,181,183..184,186..200,202..210,212,231..235,237..239,241..242,248..254,259,279..281,290,293..295,297,300..301,303,305,310..311,313,316..317,319..320,330..332,336..337,339,341,343..346,348,383..384,388,391..393,396..397,412..415,418,430..437,439,441..445,454..463,469..472,479..482,491,496,506..510,525,533,541..544,553..560,569..573,575,579,589..592,597..602,610,613,616..618,629,631..634,637,640,645..646,652..653,655,657..659,668..670,674,676,679..682} (298 alike) : DataTypeConversion  OutDataTypeStr=boolean
  UnitConverter{3..4,45,47,49,51,53,93,95,103,105,107,109,111,157,162,185,285..287,291,312,333..335,338,385,398..400,405..408,419..426,440,450..453,498..501,536..537,545..552,561..568,580..582,585..588,594..596,603..608,612,621..622,624..628,664..665,671,677,685} (98 alike) : DataTypeConversion  OutDataTypeStr=single
  UnitConverter{17..20,390,394..395} (7 alike) : DataTypeConversion  OutDataTypeStr=uint16
  UnitConverter{288,387,483..486,497,515..522,528..531} (19 alike) : DataTypeConversion  OutDataTypeStr=uint32
  VACC_HVTHCMSysAvail_enum_Inproc : FVT_lib/outp/OverrideAndLimit  SystemSampleTime=-1  VariantActivationTime=update diagram  Latency=0  AutoFrameSizeCalculation=off
      link override Signal_Limit/_maxval: Value=KOUTP_HVTHCMSysAvail_enum_maxval
      link override Signal_Limit/_minval: Value=KOUTP_HVTHCMSysAvail_enum_minval
      link override Signal_Override/_ovrdflg: Value=KOUTP_HVTHCMSysAvail_enum_ovrdflg
      link override Signal_Override/_ovrdval: Value=KOUTP_HVTHCMSysAvail_enum_ovrdval
  VACC_LVBattVoltSta_enum_Inproc : FVT_lib/outp/OverrideAndLimit  SystemSampleTime=-1  VariantActivationTime=update diagram  Latency=0  AutoFrameSizeCalculation=off
      link override Signal_Limit/_maxval: Value=KOUTP_LVBattVoltSta_enum_maxval
      link override Signal_Limit/_minval: Value=KOUTP_LVBattVoltSta_enum_minval
      link override Signal_Override/_ovrdflg: Value=KOUTP_LVBattVoltSta_enum_ovrdflg
      link override Signal_Override/_ovrdval: Value=KOUTP_LVBattVoltSta_enum_ovrdval
  VACC_VehHVPwrAvail4THCM_W_Inproc : FVT_lib/outp/OverrideAndLimit  SystemSampleTime=-1  VariantActivationTime=update diagram  Latency=0  AutoFrameSizeCalculation=off
      link override Signal_Limit/_maxval: Value=KOUTP_VehHVPwrAvail4THCM_W_maxval
      link override Signal_Limit/_minval: Value=KOUTP_VehHVPwrAvail4THCM_W_minval
      link override Signal_Override/_ovrdflg: Value=KOUTP_VehHVPwrAvail4THCM_W_ovrdflg
      link override Signal_Override/_ovrdval: Value=KOUTP_VehHVPwrAvail4THCM_W_ovrdval
  VAPM_ABSActiveTimeOut_flg_Inproc : FVT_lib/outp/OverrideAndLimit  SystemSampleTime=-1  VariantActivationTime=update diagram  Latency=0  AutoFrameSizeCalculation=off
      link override Signal_Limit/_maxval: Value=KOUTP_ABSActiveTimeOut_flg_maxval
      link override Signal_Limit/_minval: Value=KOUTP_ABSActiveTimeOut_flg_minval
      link override Signal_Override/_ovrdflg: Value=KOUTP_ABSActiveTimeOut_flg_ovrdflg
      link override Signal_Override/_ovrdval: Value=KOUTP_ABSActiveTimeOut_flg_ovrdval
  VAPM_ABSActive_flg_Inproc : FVT_lib/outp/OverrideAndLimit  SystemSampleTime=-1  VariantActivationTime=update diagram  Latency=0  AutoFrameSizeCalculation=off
      link override Signal_Limit/_maxval: Value=KOUTP_ABSActive_flg_maxval
      link override Signal_Limit/_minval: Value=KOUTP_ABSActive_flg_minval
      link override Signal_Override/_ovrdflg: Value=KOUTP_ABSActive_flg_ovrdflg
      link override Signal_Override/_ovrdval: Value=KOUTP_ABSActive_flg_ovrdval
  VAPM_APSAngleTarget_Deg_Inproc : FVT_lib/outp/OverrideAndLimit  SystemSampleTime=-1  VariantActivationTime=update diagram  Latency=0  AutoFrameSizeCalculation=off
      link override Signal_Limit/_maxval: Value=KOUTP_APSAngleTarget_Deg_maxval
      link override Signal_Limit/_minval: Value=KOUTP_APSAngleTarget_Deg_minval
      link override Signal_Override/_ovrdflg: Value=KOUTP_APSAngleTarget_Deg_ovrdflg
      link override Signal_Override/_ovrdval: Value=KOUTP_APSAngleTarget_Deg_ovrdval
  VAPM_APSDFLL_cm_Inproc : FVT_lib/outp/OverrideAndLimit  SystemSampleTime=-1  VariantActivationTime=update diagram  Latency=0  AutoFrameSizeCalculation=off
      link override Signal_Limit/_maxval: Value=KOUTP_APSDFLL_cm_maxval
      link override Signal_Limit/_minval: Value=KOUTP_APSDFLL_cm_minval
      link override Signal_Override/_ovrdflg: Value=KOUTP_APSDFLL_cm_ovrdflg
      link override Signal_Override/_ovrdval: Value=KOUTP_APSDFLL_cm_ovrdval
  VAPM_APSDFLR_cm_Inproc : FVT_lib/outp/OverrideAndLimit  SystemSampleTime=-1  VariantActivationTime=update diagram  Latency=0  AutoFrameSizeCalculation=off
      link override Signal_Limit/_maxval: Value=KOUTP_APSDFLR_cm_maxval
      link override Signal_Limit/_minval: Value=KOUTP_APSDFLR_cm_minval
      link override Signal_Override/_ovrdflg: Value=KOUTP_APSDFLR_cm_ovrdflg
      link override Signal_Override/_ovrdval: Value=KOUTP_APSDFLR_cm_ovrdval
  VAPM_APSDRLL_cm_Inproc : FVT_lib/outp/OverrideAndLimit  SystemSampleTime=-1  VariantActivationTime=update diagram  Latency=0  AutoFrameSizeCalculation=off
      link override Signal_Limit/_maxval: Value=KOUTP_APSDRLL_cm_maxval
      link override Signal_Limit/_minval: Value=KOUTP_APSDRLL_cm_minval
      link override Signal_Override/_ovrdflg: Value=KOUTP_APSDRLL_cm_ovrdflg
      link override Signal_Override/_ovrdval: Value=KOUTP_APSDRLL_cm_ovrdval
  VAPM_APSDRLR_cm_Inproc : FVT_lib/outp/OverrideAndLimit  SystemSampleTime=-1  VariantActivationTime=update diagram  Latency=0  AutoFrameSizeCalculation=off
      link override Signal_Limit/_maxval: Value=KOUTP_APSDRLR_cm_maxval
      link override Signal_Limit/_minval: Value=KOUTP_APSDRLR_cm_minval
      link override Signal_Override/_ovrdflg: Value=KOUTP_APSDRLR_cm_ovrdflg
      link override Signal_Override/_ovrdval: Value=KOUTP_APSDRLR_cm_ovrdval
  VAPM_APSExitCondition_enum_Inproc : FVT_lib/outp/OverrideAndLimit  SystemSampleTime=-1  VariantActivationTime=update diagram  Latency=0  AutoFrameSizeCalculation=off
      link override Signal_Limit/_maxval: Value=KOUTP_APSExitCondition_enum_maxval
      link override Signal_Limit/_minval: Value=KOUTP_APSExitCondition_enum_minval
      link override Signal_Override/_ovrdflg: Value=KOUTP_APSExitCondition_enum_ovrdflg
      link override Signal_Override/_ovrdval: Value=KOUTP_APSExitCondition_enum_ovrdval
  VAPM_APSHWVer_enum_Inproc : FVT_lib/outp/OverrideAndLimit  SystemSampleTime=-1  VariantActivationTime=update diagram  Latency=0  AutoFrameSizeCalculation=off
      link override Signal_Limit/_maxval: Value=KOUTP_APSHWVer_enum_maxval
      link override Signal_Limit/_minval: Value=KOUTP_APSHWVer_enum_minval
      link override Signal_Override/_ovrdflg: Value=KOUTP_APSHWVer_enum_ovrdflg
      link override Signal_Override/_ovrdval: Value=KOUTP_APSHWVer_enum_ovrdval
  VAPM_APSProgressPCT_pct_Inproc : FVT_lib/outp/OverrideAndLimit  SystemSampleTime=-1  VariantActivationTime=update diagram  Latency=0  AutoFrameSizeCalculation=off
      link override Signal_Limit/_maxval: Value=KOUTP_APSProgressPCT_pct_maxval
      link override Signal_Limit/_minval: Value=KOUTP_APSProgressPCT_pct_minval
      link override Signal_Override/_ovrdflg: Value=KOUTP_APSProgressPCT_pct_ovrdflg
      link override Signal_Override/_ovrdval: Value=KOUTP_APSProgressPCT_pct_ovrdval
  VAPM_APSRQDisplay_enum_Inproc : FVT_lib/outp/OverrideAndLimit  SystemSampleTime=-1  VariantActivationTime=update diagram  Latency=0  AutoFrameSizeCalculation=off
      link override Signal_Limit/_maxval: Value=KOUTP_APSRQDisplay_enum_maxval
      link override Signal_Limit/_minval: Value=KOUTP_APSRQDisplay_enum_minval
      link override Signal_Override/_ovrdflg: Value=KOUTP_APSRQDisplay_enum_ovrdflg
      link override Signal_Override/_ovrdval: Value=KOUTP_APSRQDisplay_enum_ovrdval
  VAPM_APSRqEPASCtrl_flg_Inproc : FVT_lib/outp/OverrideAndLimit  SystemSampleTime=-1  VariantActivationTime=update diagram  Latency=0  AutoFrameSizeCalculation=off
      link override Signal_Limit/_maxval: Value=KOUTP_APSRqEPASCtrl_flg_maxval
      link override Signal_Limit/_minval: Value=KOUTP_APSRqEPASCtrl_flg_minval
      link override Signal_Override/_ovrdflg: Value=KOUTP_APSRqEPASCtrl_flg_ovrdflg
      link override Signal_Override/_ovrdval: Value=KOUTP_APSRqEPASCtrl_flg_ovrdval
  VAPM_APSSWVer_enum_Inproc : FVT_lib/outp/OverrideAndLimit  SystemSampleTime=-1  VariantActivationTime=update diagram  Latency=0  AutoFrameSizeCalculation=off
      link override Signal_Limit/_maxval: Value=KOUTP_APSSWVer_enum_maxval
      link override Signal_Limit/_minval: Value=KOUTP_APSSWVer_enum_minval
      link override Signal_Override/_ovrdflg: Value=KOUTP_APSSWVer_enum_ovrdflg
      link override Signal_Override/_ovrdval: Value=KOUTP_APSSWVer_enum_ovrdval
  VAPM_APSVRqEPASCtrl_flg_Inproc : FVT_lib/outp/OverrideAndLimit  SystemSampleTime=-1  VariantActivationTime=update diagram  Latency=0  AutoFrameSizeCalculation=off
      link override Signal_Limit/_maxval: Value=KOUTP_APSVRqEPASCtrl_flg_maxval
      link override Signal_Limit/_minval: Value=KOUTP_APSVRqEPASCtrl_flg_minval
      link override Signal_Override/_ovrdflg: Value=KOUTP_APSVRqEPASCtrl_flg_ovrdflg
      link override Signal_Override/_ovrdval: Value=KOUTP_APSVRqEPASCtrl_flg_ovrdval
  VAPM_AVMErrSTATimeOut_flg_Inproc : FVT_lib/outp/OverrideAndLimit  SystemSampleTime=-1  VariantActivationTime=update diagram  Latency=0  AutoFrameSizeCalculation=off
      link override Signal_Limit/_maxval: Value=KOUTP_AVMErrSTATimeOut_flg_maxval
      link override Signal_Limit/_minval: Value=KOUTP_AVMErrSTATimeOut_flg_minval
      link override Signal_Override/_ovrdflg: Value=KOUTP_AVMErrSTATimeOut_flg_ovrdflg
      link override Signal_Override/_ovrdval: Value=KOUTP_AVMErrSTATimeOut_flg_ovrdval
  VAPM_AVMErrSTA_flg_Inproc : FVT_lib/outp/OverrideAndLimit  SystemSampleTime=-1  VariantActivationTime=update diagram  Latency=0  AutoFrameSizeCalculation=off
      link override Signal_Limit/_maxval: Value=KOUTP_AVMErrSTA_flg_maxval
      link override Signal_Limit/_minval: Value=KOUTP_AVMErrSTA_flg_minval
      link override Signal_Override/_ovrdflg: Value=KOUTP_AVMErrSTA_flg_ovrdflg
      link override Signal_Override/_ovrdval: Value=KOUTP_AVMErrSTA_flg_ovrdval
  VAPM_AVMParkingmodeTimeOut_flg_Inproc : FVT_lib/outp/OverrideAndLimit  SystemSampleTime=-1  VariantActivationTime=update diagram  Latency=0  AutoFrameSizeCalculation=off
      link override Signal_Limit/_maxval: Value=KOUTP_AVMParkingmodeTimeOut_flg_maxval
      link override Signal_Limit/_minval: Value=KOUTP_AVMParkingmodeTimeOut_flg_minval
      link override Signal_Override/_ovrdflg: Value=KOUTP_AVMParkingmodeTimeOut_flg_ovrdflg
      link override Signal_Override/_ovrdval: Value=KOUTP_AVMParkingmodeTimeOut_flg_ovrdval
  VAPM_AVMParkingmode_enum_Inproc : FVT_lib/outp/OverrideAndLimit  SystemSampleTime=-1  VariantActivationTime=update diagram  Latency=0  AutoFrameSizeCalculation=off
      link override Signal_Limit/_maxval: Value=KOUTP_AVMParkingmode_enum_maxval
      link override Signal_Limit/_minval: Value=KOUTP_AVMParkingmode_enum_minval
      link override Signal_Override/_ovrdflg: Value=KOUTP_AVMParkingmode_enum_ovrdflg
      link override Signal_Override/_ovrdval: Value=KOUTP_AVMParkingmode_enum_ovrdval
  VAPM_AVMparkingcancelTimeOut_flg_Inproc : FVT_lib/outp/OverrideAndLimit  SystemSampleTime=-1  VariantActivationTime=update diagram  Latency=0  AutoFrameSizeCalculation=off
      link override Signal_Limit/_maxval: Value=KOUTP_AVMparkingcancelTimeOut_flg_maxval
      link override Signal_Limit/_minval: Value=KOUTP_AVMparkingcancelTimeOut_flg_minval
      link override Signal_Override/_ovrdflg: Value=KOUTP_AVMparkingcancelTimeOut_flg_ovrdflg
      link override Signal_Override/_ovrdval: Value=KOUTP_AVMparkingcancelTimeOut_flg_ovrdval
  VAPM_AVMparkingcancel_enum_Inproc : FVT_lib/outp/OverrideAndLimit  SystemSampleTime=-1  VariantActivationTime=update diagram  Latency=0  AutoFrameSizeCalculation=off
      link override Signal_Limit/_maxval: Value=KOUTP_AVMparkingcancel_enum_maxval
      link override Signal_Limit/_minval: Value=KOUTP_AVMparkingcancel_enum_minval
      link override Signal_Override/_ovrdflg: Value=KOUTP_AVMparkingcancel_enum_ovrdflg
      link override Signal_Override/_ovrdval: Value=KOUTP_AVMparkingcancel_enum_ovrdval
  VAPM_AVMparkingexcuteTimeOut_flg_Inproc : FVT_lib/outp/OverrideAndLimit  SystemSampleTime=-1  VariantActivationTime=update diagram  Latency=0  AutoFrameSizeCalculation=off
      link override Signal_Limit/_maxval: Value=KOUTP_AVMparkingexcuteTimeOut_flg_maxval
      link override Signal_Limit/_minval: Value=KOUTP_AVMparkingexcuteTimeOut_flg_minval
      link override Signal_Override/_ovrdflg: Value=KOUTP_AVMparkingexcuteTimeOut_flg_ovrdflg
      link override Signal_Override/_ovrdval: Value=KOUTP_AVMparkingexcuteTimeOut_flg_ovrdval
  VAPM_AVMparkingexcute_enum_Inproc : FVT_lib/outp/OverrideAndLimit  SystemSampleTime=-1  VariantActivationTime=update diagram  Latency=0  AutoFrameSizeCalculation=off
      link override Signal_Limit/_maxval: Value=KOUTP_AVMparkingexcute_enum_maxval
      link override Signal_Limit/_minval: Value=KOUTP_AVMparkingexcute_enum_minval
      link override Signal_Override/_ovrdflg: Value=KOUTP_AVMparkingexcute_enum_ovrdflg
      link override Signal_Override/_ovrdval: Value=KOUTP_AVMparkingexcute_enum_ovrdval
  VAPM_BrkPedalPosTimeOut_flg_Inproc : FVT_lib/outp/OverrideAndLimit  SystemSampleTime=-1  VariantActivationTime=update diagram  Latency=0  AutoFrameSizeCalculation=off
      link override Signal_Limit/_maxval: Value=KOUTP_BrkPedalPosTimeOut_flg_maxval
      link override Signal_Limit/_minval: Value=KOUTP_BrkPedalPosTimeOut_flg_minval
      link override Signal_Override/_ovrdflg: Value=KOUTP_BrkPedalPosTimeOut_flg_ovrdflg
      link override Signal_Override/_ovrdval: Value=KOUTP_BrkPedalPosTimeOut_flg_ovrdval
  VAPM_BrkPedalPos_pct_Inproc : FVT_lib/outp/OverrideAndLimit  SystemSampleTime=-1  VariantActivationTime=update diagram  Latency=0  AutoFrameSizeCalculation=off
      link override Signal_Limit/_maxval: Value=KOUTP_BrkPedalPos_pct_maxval
      link override Signal_Limit/_minval: Value=KOUTP_BrkPedalPos_pct_minval
      link override Signal_Override/_ovrdflg: Value=KOUTP_BrkPedalPos_pct_ovrdflg
      link override Signal_Override/_ovrdval: Value=KOUTP_BrkPedalPos_pct_ovrdval
  VAPM_BrkSwStaTimeOut_flg_Inproc : FVT_lib/outp/OverrideAndLimit  SystemSampleTime=-1  VariantActivationTime=update diagram  Latency=0  AutoFrameSizeCalculation=off
      link override Signal_Limit/_maxval: Value=KOUTP_BrkSwStaTimeOut_flg_maxval
      link override Signal_Limit/_minval: Value=KOUTP_BrkSwStaTimeOut_flg_minval
      link override Signal_Override/_ovrdflg: Value=KOUTP_BrkSwStaTimeOut_flg_ovrdflg
      link override Signal_Override/_ovrdval: Value=KOUTP_BrkSwStaTimeOut_flg_ovrdval
  VAPM_BrkSwSta_flg_Inproc : FVT_lib/outp/OverrideAndLimit  SystemSampleTime=-1  VariantActivationTime=update diagram  Latency=0  AutoFrameSizeCalculation=off
      link override Signal_Limit/_maxval: Value=KOUTP_BrkSwSta_flg_maxval
      link override Signal_Limit/_minval: Value=KOUTP_BrkSwSta_flg_minval
      link override Signal_Override/_ovrdflg: Value=KOUTP_BrkSwSta_flg_ovrdflg
      link override Signal_Override/_ovrdval: Value=KOUTP_BrkSwSta_flg_ovrdval
  VAPM_BrkSwVTimeOut_flg_Inproc : FVT_lib/outp/OverrideAndLimit  SystemSampleTime=-1  VariantActivationTime=update diagram  Latency=0  AutoFrameSizeCalculation=off
      link override Signal_Limit/_maxval: Value=KOUTP_BrkSwVTimeOut_flg_maxval
      link override Signal_Limit/_minval: Value=KOUTP_BrkSwVTimeOut_flg_minval
      link override Signal_Override/_ovrdflg: Value=KOUTP_BrkSwVTimeOut_flg_ovrdflg
      link override Signal_Override/_ovrdval: Value=KOUTP_BrkSwVTimeOut_flg_ovrdval
  VAPM_BrkSwV_flg_Inproc : FVT_lib/outp/OverrideAndLimit  SystemSampleTime=-1  VariantActivationTime=update diagram  Latency=0  AutoFrameSizeCalculation=off
      link override Signal_Limit/_maxval: Value=KOUTP_BrkSwV_flg_maxval
      link override Signal_Limit/_minval: Value=KOUTP_BrkSwV_flg_minval
      link override Signal_Override/_ovrdflg: Value=KOUTP_BrkSwV_flg_ovrdflg
      link override Signal_Override/_ovrdval: Value=KOUTP_BrkSwV_flg_ovrdval
  VAPM_CAASSta_enum_Inproc : FVT_lib/outp/OverrideAndLimit  SystemSampleTime=-1  VariantActivationTime=update diagram  Latency=0  AutoFrameSizeCalculation=off
      link override Signal_Limit/_maxval: Value=KOUTP_CAASSta_enum_maxval
      link override Signal_Limit/_minval: Value=KOUTP_CAASSta_enum_minval
      link override Signal_Override/_ovrdflg: Value=KOUTP_CAASSta_enum_ovrdflg
      link override Signal_Override/_ovrdval: Value=KOUTP_CAASSta_enum_ovrdval
  VAPM_CAASSwTimeOut_flg_Inproc : FVT_lib/outp/OverrideAndLimit  SystemSampleTime=-1  VariantActivationTime=update diagram  Latency=0  AutoFrameSizeCalculation=off
      link override Signal_Limit/_maxval: Value=KOUTP_CAASSwTimeOut_flg_maxval
      link override Signal_Limit/_minval: Value=KOUTP_CAASSwTimeOut_flg_minval
      link override Signal_Override/_ovrdflg: Value=KOUTP_CAASSwTimeOut_flg_ovrdflg
      link override Signal_Override/_ovrdval: Value=KOUTP_CAASSwTimeOut_flg_ovrdval
  VAPM_CAASSw_enum_Inproc : FVT_lib/outp/OverrideAndLimit  SystemSampleTime=-1  VariantActivationTime=update diagram  Latency=0  AutoFrameSizeCalculation=off
      link override Signal_Limit/_maxval: Value=KOUTP_CAASSw_enum_maxval
      link override Signal_Limit/_minval: Value=KOUTP_CAASSw_enum_minval
      link override Signal_Override/_ovrdflg: Value=KOUTP_CAASSw_enum_ovrdflg
      link override Signal_Override/_ovrdval: Value=KOUTP_CAASSw_enum_ovrdval
  VAPM_Chime_enum_Inproc : FVT_lib/outp/OverrideAndLimit  SystemSampleTime=-1  VariantActivationTime=update diagram  Latency=0  AutoFrameSizeCalculation=off
      link override Signal_Limit/_maxval: Value=KOUTP_Chime_enum_maxval
      link override Signal_Limit/_minval: Value=KOUTP_Chime_enum_minval
      link override Signal_Override/_ovrdflg: Value=KOUTP_Chime_enum_ovrdflg
      link override Signal_Override/_ovrdval: Value=KOUTP_Chime_enum_ovrdval
  VAPM_ChrgPlugSta_enum_Inproc : FVT_lib/outp/OverrideAndLimit  SystemSampleTime=-1  VariantActivationTime=update diagram  Latency=0  AutoFrameSizeCalculation=off
      link override Signal_Limit/_maxval: Value=KOUTP_ChrgPlugSta_enum_maxval
      link override Signal_Limit/_minval: Value=KOUTP_ChrgPlugSta_enum_minval
      link override Signal_Override/_ovrdflg: Value=KOUTP_ChrgPlugSta_enum_ovrdflg
      link override Signal_Override/_ovrdval: Value=KOUTP_ChrgPlugSta_enum_ovrdval
  VAPM_DriIntendTimeOut_flg_Inproc : FVT_lib/outp/OverrideAndLimit  SystemSampleTime=-1  VariantActivationTime=update diagram  Latency=0  AutoFrameSizeCalculation=off
      link override Signal_Limit/_maxval: Value=KOUTP_DriIntendTimeOut_flg_maxval
      link override Signal_Limit/_minval: Value=KOUTP_DriIntendTimeOut_flg_minval
      link override Signal_Override/_ovrdflg: Value=KOUTP_DriIntendTimeOut_flg_ovrdflg
      link override Signal_Override/_ovrdval: Value=KOUTP_DriIntendTimeOut_flg_ovrdval
  VAPM_DriIntend_enum_Inproc : FVT_lib/outp/OverrideAndLimit  SystemSampleTime=-1  VariantActivationTime=update diagram  Latency=0  AutoFrameSizeCalculation=off
      link override Signal_Limit/_maxval: Value=KOUTP_DriIntend_enum_maxval
      link override Signal_Limit/_minval: Value=KOUTP_DriIntend_enum_minval
      link override Signal_Override/_ovrdflg: Value=KOUTP_DriIntend_enum_ovrdflg
      link override Signal_Override/_ovrdval: Value=KOUTP_DriIntend_enum_ovrdval
  VAPM_DriverSeatBeltCmdTimeOut_flg_Inproc : FVT_lib/outp/OverrideAndLimit  SystemSampleTime=-1  VariantActivationTime=update diagram  Latency=0  AutoFrameSizeCalculation=off
      link override Signal_Limit/_maxval: Value=KOUTP_DriverSeatBeltCmdTimeOut_flg_maxval
      link override Signal_Limit/_minval: Value=KOUTP_DriverSeatBeltCmdTimeOut_flg_minval
      link override Signal_Override/_ovrdflg: Value=KOUTP_DriverSeatBeltCmdTimeOut_flg_ovrdflg
      link override Signal_Override/_ovrdval: Value=KOUTP_DriverSeatBeltCmdTimeOut_flg_ovrdval
  VAPM_DriverSeatBeltCmd_flg_Inproc : FVT_lib/outp/OverrideAndLimit  SystemSampleTime=-1  VariantActivationTime=update diagram  Latency=0  AutoFrameSizeCalculation=off
      link override Signal_Limit/_maxval: Value=KOUTP_DriverSeatBeltCmd_flg_maxval
      link override Signal_Limit/_minval: Value=KOUTP_DriverSeatBeltCmd_flg_minval
      link override Signal_Override/_ovrdflg: Value=KOUTP_DriverSeatBeltCmd_flg_ovrdflg
      link override Signal_Override/_ovrdval: Value=KOUTP_DriverSeatBeltCmd_flg_ovrdval
  VAPM_EPBErrStaTimeOut_flg_Inproc : FVT_lib/outp/OverrideAndLimit  SystemSampleTime=-1  VariantActivationTime=update diagram  Latency=0  AutoFrameSizeCalculation=off
      link override Signal_Limit/_maxval: Value=KOUTP_EPBErrStaTimeOut_flg_maxval
      link override Signal_Limit/_minval: Value=KOUTP_EPBErrStaTimeOut_flg_minval
      link override Signal_Override/_ovrdflg: Value=KOUTP_EPBErrStaTimeOut_flg_ovrdflg
      link override Signal_Override/_ovrdval: Value=KOUTP_EPBErrStaTimeOut_flg_ovrdval
  VAPM_EPBErrSta_enum_Inproc : FVT_lib/outp/OverrideAndLimit  SystemSampleTime=-1  VariantActivationTime=update diagram  Latency=0  AutoFrameSizeCalculation=off
      link override Signal_Limit/_maxval: Value=KOUTP_EPBErrSta_enum_maxval
      link override Signal_Limit/_minval: Value=KOUTP_EPBErrSta_enum_minval
      link override Signal_Override/_ovrdflg: Value=KOUTP_EPBErrSta_enum_ovrdflg
      link override Signal_Override/_ovrdval: Value=KOUTP_EPBErrSta_enum_ovrdval
  VAPM_EPBExtApplyAvailTimeOut_flg_Inproc : FVT_lib/outp/OverrideAndLimit  SystemSampleTime=-1  VariantActivationTime=update diagram  Latency=0  AutoFrameSizeCalculation=off
      link override Signal_Limit/_maxval: Value=KOUTP_EPBExtApplyAvailTimeOut_flg_maxval
      link override Signal_Limit/_minval: Value=KOUTP_EPBExtApplyAvailTimeOut_flg_minval
      link override Signal_Override/_ovrdflg: Value=KOUTP_EPBExtApplyAvailTimeOut_flg_ovrdflg
      link override Signal_Override/_ovrdval: Value=KOUTP_EPBExtApplyAvailTimeOut_flg_ovrdval
  VAPM_EPBExtApplyAvail_flg_Inproc : FVT_lib/outp/OverrideAndLimit  SystemSampleTime=-1  VariantActivationTime=update diagram  Latency=0  AutoFrameSizeCalculation=off
      link override Signal_Limit/_maxval: Value=KOUTP_EPBExtApplyAvail_flg_maxval
      link override Signal_Limit/_minval: Value=KOUTP_EPBExtApplyAvail_flg_minval
      link override Signal_Override/_ovrdflg: Value=KOUTP_EPBExtApplyAvail_flg_ovrdflg
      link override Signal_Override/_ovrdval: Value=KOUTP_EPBExtApplyAvail_flg_ovrdval
  VAPM_EPBExtReleaseAvailTimeOut_flg_Inproc : FVT_lib/outp/OverrideAndLimit  SystemSampleTime=-1  VariantActivationTime=update diagram  Latency=0  AutoFrameSizeCalculation=off
      link override Signal_Limit/_maxval: Value=KOUTP_EPBExtReleaseAvailTimeOut_flg_maxval
      link override Signal_Limit/_minval: Value=KOUTP_EPBExtReleaseAvailTimeOut_flg_minval
      link override Signal_Override/_ovrdflg: Value=KOUTP_EPBExtReleaseAvailTimeOut_flg_ovrdflg
      link override Signal_Override/_ovrdval: Value=KOUTP_EPBExtReleaseAvailTimeOut_flg_ovrdval
  VAPM_EPBExtReleaseAvail_flg_Inproc : FVT_lib/outp/OverrideAndLimit  SystemSampleTime=-1  VariantActivationTime=update diagram  Latency=0  AutoFrameSizeCalculation=off
      link override Signal_Limit/_maxval: Value=KOUTP_EPBExtReleaseAvail_flg_maxval
      link override Signal_Limit/_minval: Value=KOUTP_EPBExtReleaseAvail_flg_minval
      link override Signal_Override/_ovrdflg: Value=KOUTP_EPBExtReleaseAvail_flg_ovrdflg
      link override Signal_Override/_ovrdval: Value=KOUTP_EPBExtReleaseAvail_flg_ovrdval
  VAPM_EPBStaTimeOut_flg_Inproc : FVT_lib/outp/OverrideAndLimit  SystemSampleTime=-1  VariantActivationTime=update diagram  Latency=0  AutoFrameSizeCalculation=off
      link override Signal_Limit/_maxval: Value=KOUTP_EPBStaTimeOut_flg_maxval
      link override Signal_Limit/_minval: Value=KOUTP_EPBStaTimeOut_flg_minval
      link override Signal_Override/_ovrdflg: Value=KOUTP_EPBStaTimeOut_flg_ovrdflg
      link override Signal_Override/_ovrdval: Value=KOUTP_EPBStaTimeOut_flg_ovrdval
  VAPM_EPBSta_enum_Inproc : FVT_lib/outp/OverrideAndLimit  SystemSampleTime=-1  VariantActivationTime=update diagram  Latency=0  AutoFrameSizeCalculation=off
      link override Signal_Limit/_maxval: Value=KOUTP_EPBSta_enum_maxval
      link override Signal_Limit/_minval: Value=KOUTP_EPBSta_enum_minval
      link override Signal_Override/_ovrdflg: Value=KOUTP_EPBSta_enum_ovrdflg
      link override Signal_Override/_ovrdval: Value=KOUTP_EPBSta_enum_ovrdval
  VAPM_EPSAOIControlTimeOut_flg_Inproc : FVT_lib/outp/OverrideAndLimit  SystemSampleTime=-1  VariantActivationTime=update diagram  Latency=0  AutoFrameSizeCalculation=off
      link override Signal_Limit/_maxval: Value=KOUTP_EPSAOIControlTimeOut_flg_maxval
      link override Signal_Limit/_minval: Value=KOUTP_EPSAOIControlTimeOut_flg_minval
      link override Signal_Override/_ovrdflg: Value=KOUTP_EPSAOIControlTimeOut_flg_ovrdflg
      link override Signal_Override/_ovrdval: Value=KOUTP_EPSAOIControlTimeOut_flg_ovrdval
  VAPM_EPSAOIControl_enum_Inproc : FVT_lib/outp/OverrideAndLimit  SystemSampleTime=-1  VariantActivationTime=update diagram  Latency=0  AutoFrameSizeCalculation=off
      link override Signal_Limit/_maxval: Value=KOUTP_EPSAOIControl_enum_maxval
      link override Signal_Limit/_minval: Value=KOUTP_EPSAOIControl_enum_minval
      link override Signal_Override/_ovrdflg: Value=KOUTP_EPSAOIControl_enum_ovrdflg
      link override Signal_Override/_ovrdval: Value=KOUTP_EPSAOIControl_enum_ovrdval
  VAPM_ESCAPSStaTimeOut_flg_Inproc : FVT_lib/outp/OverrideAndLimit  SystemSampleTime=-1  VariantActivationTime=update diagram  Latency=0  AutoFrameSizeCalculation=off
      link override Signal_Limit/_maxval: Value=KOUTP_ESCAPSStaTimeOut_flg_maxval
      link override Signal_Limit/_minval: Value=KOUTP_ESCAPSStaTimeOut_flg_minval
      link override Signal_Override/_ovrdflg: Value=KOUTP_ESCAPSStaTimeOut_flg_ovrdflg
      link override Signal_Override/_ovrdval: Value=KOUTP_ESCAPSStaTimeOut_flg_ovrdval
  VAPM_ESCAPSSta_enum_Inproc : FVT_lib/outp/OverrideAndLimit  SystemSampleTime=-1  VariantActivationTime=update diagram  Latency=0  AutoFrameSizeCalculation=off
      link override Signal_Limit/_maxval: Value=KOUTP_ESCAPSSta_enum_maxval
      link override Signal_Limit/_minval: Value=KOUTP_ESCAPSSta_enum_minval
      link override Signal_Override/_ovrdflg: Value=KOUTP_ESCAPSSta_enum_ovrdflg
      link override Signal_Override/_ovrdval: Value=KOUTP_ESCAPSSta_enum_ovrdval
  VAPM_ESCStandstillTimeOut_flg_Inproc : FVT_lib/outp/OverrideAndLimit  SystemSampleTime=-1  VariantActivationTime=update diagram  Latency=0  AutoFrameSizeCalculation=off
      link override Signal_Limit/_maxval: Value=KOUTP_ESCStandstillTimeOut_flg_maxval
      link override Signal_Limit/_minval: Value=KOUTP_ESCStandstillTimeOut_flg_minval
      link override Signal_Override/_ovrdflg: Value=KOUTP_ESCStandstillTimeOut_flg_ovrdflg
      link override Signal_Override/_ovrdval: Value=KOUTP_ESCStandstillTimeOut_flg_ovrdval
  VAPM_ESCStandstill_flg_Inproc : FVT_lib/outp/OverrideAndLimit  SystemSampleTime=-1  VariantActivationTime=update diagram  Latency=0  AutoFrameSizeCalculation=off
      link override Signal_Limit/_maxval: Value=KOUTP_ESCStandstill_flg_maxval
      link override Signal_Limit/_minval: Value=KOUTP_ESCStandstill_flg_minval
      link override Signal_Override/_ovrdflg: Value=KOUTP_ESCStandstill_flg_ovrdflg
      link override Signal_Override/_ovrdval: Value=KOUTP_ESCStandstill_flg_ovrdval
  VAPM_FSOffSwTimeOut_flg_Inproc : FVT_lib/outp/OverrideAndLimit  SystemSampleTime=-1  VariantActivationTime=update diagram  Latency=0  AutoFrameSizeCalculation=off
      link override Signal_Limit/_maxval: Value=KOUTP_FSOffSwTimeOut_flg_maxval
      link override Signal_Limit/_minval: Value=KOUTP_FSOffSwTimeOut_flg_minval
      link override Signal_Override/_ovrdflg: Value=KOUTP_FSOffSwTimeOut_flg_ovrdflg
      link override Signal_Override/_ovrdval: Value=KOUTP_FSOffSwTimeOut_flg_ovrdval
  VAPM_FSOffSw_enum_Inproc : FVT_lib/outp/OverrideAndLimit  SystemSampleTime=-1  VariantActivationTime=update diagram  Latency=0  AutoFrameSizeCalculation=off
      link override Signal_Limit/_maxval: Value=KOUTP_FSOffSw_enum_maxval
      link override Signal_Limit/_minval: Value=KOUTP_FSOffSw_enum_minval
      link override Signal_Override/_ovrdflg: Value=KOUTP_FSOffSw_enum_ovrdflg
      link override Signal_Override/_ovrdval: Value=KOUTP_FSOffSw_enum_ovrdval
  VAPM_GRADETimeOut_flg_Inproc : FVT_lib/outp/OverrideAndLimit  SystemSampleTime=-1  VariantActivationTime=update diagram  Latency=0  AutoFrameSizeCalculation=off
      link override Signal_Limit/_maxval: Value=KOUTP_GRADETimeOut_flg_maxval
      link override Signal_Limit/_minval: Value=KOUTP_GRADETimeOut_flg_minval
      link override Signal_Override/_ovrdflg: Value=KOUTP_GRADETimeOut_flg_ovrdflg
      link override Signal_Override/_ovrdval: Value=KOUTP_GRADETimeOut_flg_ovrdval
  VAPM_GRADE_Deg_Inproc : FVT_lib/outp/OverrideAndLimit  SystemSampleTime=-1  VariantActivationTime=update diagram  Latency=0  AutoFrameSizeCalculation=off
      link override Signal_Limit/_maxval: Value=KOUTP_GRADE_Deg_maxval
      link override Signal_Limit/_minval: Value=KOUTP_GRADE_Deg_minval
      link override Signal_Override/_ovrdflg: Value=KOUTP_GRADE_Deg_ovrdflg
      link override Signal_Override/_ovrdval: Value=KOUTP_GRADE_Deg_ovrdval
  VAPM_IVIScreenTimeOut_flg_Inproc : FVT_lib/outp/OverrideAndLimit  SystemSampleTime=-1  VariantActivationTime=update diagram  Latency=0  AutoFrameSizeCalculation=off
      link override Signal_Limit/_maxval: Value=KOUTP_IVIScreenTimeOut_flg_maxval
      link override Signal_Limit/_minval: Value=KOUTP_IVIScreenTimeOut_flg_minval
      link override Signal_Override/_ovrdflg: Value=KOUTP_IVIScreenTimeOut_flg_ovrdflg
      link override Signal_Override/_ovrdval: Value=KOUTP_IVIScreenTimeOut_flg_ovrdval
  VAPM_IVIScreen_enum_Inproc : FVT_lib/outp/OverrideAndLimit  SystemSampleTime=-1  VariantActivationTime=update diagram  Latency=0  AutoFrameSizeCalculation=off
      link override Signal_Limit/_maxval: Value=KOUTP_IVIScreen_enum_maxval
      link override Signal_Limit/_minval: Value=KOUTP_IVIScreen_enum_minval
      link override Signal_Override/_ovrdflg: Value=KOUTP_IVIScreen_enum_ovrdflg
      link override Signal_Override/_ovrdval: Value=KOUTP_IVIScreen_enum_ovrdval
  VAPM_IVIStatusTimeOut_flg_Inproc : FVT_lib/outp/OverrideAndLimit  SystemSampleTime=-1  VariantActivationTime=update diagram  Latency=0  AutoFrameSizeCalculation=off
      link override Signal_Limit/_maxval: Value=KOUTP_IVIStatusTimeOut_flg_maxval
      link override Signal_Limit/_minval: Value=KOUTP_IVIStatusTimeOut_flg_minval
      link override Signal_Override/_ovrdflg: Value=KOUTP_IVIStatusTimeOut_flg_ovrdflg
      link override Signal_Override/_ovrdval: Value=KOUTP_IVIStatusTimeOut_flg_ovrdval
  VAPM_IVIStatus_flg_Inproc : FVT_lib/outp/OverrideAndLimit  SystemSampleTime=-1  VariantActivationTime=update diagram  Latency=0  AutoFrameSizeCalculation=off
      link override Signal_Limit/_maxval: Value=KOUTP_IVIStatus_flg_maxval
      link override Signal_Limit/_minval: Value=KOUTP_IVIStatus_flg_minval
      link override Signal_Override/_ovrdflg: Value=KOUTP_IVIStatus_flg_ovrdflg
      link override Signal_Override/_ovrdval: Value=KOUTP_IVIStatus_flg_ovrdval
  VAPM_LFPulseCountTimeOut_flg_Inproc : FVT_lib/outp/OverrideAndLimit  SystemSampleTime=-1  VariantActivationTime=update diagram  Latency=0  AutoFrameSizeCalculation=off
      link override Signal_Limit/_maxval: Value=KOUTP_LFPulseCountTimeOut_flg_maxval
      link override Signal_Limit/_minval: Value=KOUTP_LFPulseCountTimeOut_flg_minval
      link override Signal_Override/_ovrdflg: Value=KOUTP_LFPulseCountTimeOut_flg_ovrdflg
      link override Signal_Override/_ovrdval: Value=KOUTP_LFPulseCountTimeOut_flg_ovrdval
  VAPM_LFPulseCountVTimeOut_flg_Inproc : FVT_lib/outp/OverrideAndLimit  SystemSampleTime=-1  VariantActivationTime=update diagram  Latency=0  AutoFrameSizeCalculation=off
      link override Signal_Limit/_maxval: Value=KOUTP_LFPulseCountVTimeOut_flg_maxval
      link override Signal_Limit/_minval: Value=KOUTP_LFPulseCountVTimeOut_flg_minval
      link override Signal_Override/_ovrdflg: Value=KOUTP_LFPulseCountVTimeOut_flg_ovrdflg
      link override Signal_Override/_ovrdval: Value=KOUTP_LFPulseCountVTimeOut_flg_ovrdval
  VAPM_LFPulseCountV_flg_Inproc : FVT_lib/outp/OverrideAndLimit  SystemSampleTime=-1  VariantActivationTime=update diagram  Latency=0  AutoFrameSizeCalculation=off
      link override Signal_Limit/_maxval: Value=KOUTP_LFPulseCountV_flg_maxval
      link override Signal_Limit/_minval: Value=KOUTP_LFPulseCountV_flg_minval
      link override Signal_Override/_ovrdflg: Value=KOUTP_LFPulseCountV_flg_ovrdflg
      link override Signal_Override/_ovrdval: Value=KOUTP_LFPulseCountV_flg_ovrdval
  VAPM_LFPulseCount_enum_Inproc : FVT_lib/outp/OverrideAndLimit  SystemSampleTime=-1  VariantActivationTime=update diagram  Latency=0  AutoFrameSizeCalculation=off
      link override Signal_Limit/_maxval: Value=KOUTP_LFPulseCount_enum_maxval
      link override Signal_Limit/_minval: Value=KOUTP_LFPulseCount_enum_minval
      link override Signal_Override/_ovrdflg: Value=KOUTP_LFPulseCount_enum_ovrdflg
      link override Signal_Override/_ovrdval: Value=KOUTP_LFPulseCount_enum_ovrdval
  VAPM_LFRawWhlSpeedTimeOut_flg_Inproc : FVT_lib/outp/OverrideAndLimit  SystemSampleTime=-1  VariantActivationTime=update diagram  Latency=0  AutoFrameSizeCalculation=off
      link override Signal_Limit/_maxval: Value=KOUTP_LFRawWhlSpeedTimeOut_flg_maxval
      link override Signal_Limit/_minval: Value=KOUTP_LFRawWhlSpeedTimeOut_flg_minval
      link override Signal_Override/_ovrdflg: Value=KOUTP_LFRawWhlSpeedTimeOut_flg_ovrdflg
      link override Signal_Override/_ovrdval: Value=KOUTP_LFRawWhlSpeedTimeOut_flg_ovrdval
  VAPM_LFRawWhlSpeedVTimeOut_flg_Inproc : FVT_lib/outp/OverrideAndLimit  SystemSampleTime=-1  VariantActivationTime=update diagram  Latency=0  AutoFrameSizeCalculation=off
      link override Signal_Limit/_maxval: Value=KOUTP_LFRawWhlSpeedVTimeOut_flg_maxval
      link override Signal_Limit/_minval: Value=KOUTP_LFRawWhlSpeedVTimeOut_flg_minval
      link override Signal_Override/_ovrdflg: Value=KOUTP_LFRawWhlSpeedVTimeOut_flg_ovrdflg
      link override Signal_Override/_ovrdval: Value=KOUTP_LFRawWhlSpeedVTimeOut_flg_ovrdval
  VAPM_LFRawWhlSpeedV_flg_Inproc : FVT_lib/outp/OverrideAndLimit  SystemSampleTime=-1  VariantActivationTime=update diagram  Latency=0  AutoFrameSizeCalculation=off
      link override Signal_Limit/_maxval: Value=KOUTP_LFRawWhlSpeedV_flg_maxval
      link override Signal_Limit/_minval: Value=KOUTP_LFRawWhlSpeedV_flg_minval
      link override Signal_Override/_ovrdflg: Value=KOUTP_LFRawWhlSpeedV_flg_ovrdflg
      link override Signal_Override/_ovrdval: Value=KOUTP_LFRawWhlSpeedV_flg_ovrdval
  VAPM_LFRawWhlSpeed_kph_Inproc : FVT_lib/outp/OverrideAndLimit  SystemSampleTime=-1  VariantActivationTime=update diagram  Latency=0  AutoFrameSizeCalculation=off
      link override Signal_Limit/_maxval: Value=KOUTP_LFRawWhlSpeed_kph_maxval
      link override Signal_Limit/_minval: Value=KOUTP_LFRawWhlSpeed_kph_minval
      link override Signal_Override/_ovrdflg: Value=KOUTP_LFRawWhlSpeed_kph_ovrdflg
      link override Signal_Override/_ovrdval: Value=KOUTP_LFRawWhlSpeed_kph_ovrdval
  VAPM_LFWhlRotDirTimeOut_flg_Inproc : FVT_lib/outp/OverrideAndLimit  SystemSampleTime=-1  VariantActivationTime=update diagram  Latency=0  AutoFrameSizeCalculation=off
      link override Signal_Limit/_maxval: Value=KOUTP_LFWhlRotDirTimeOut_flg_maxval
      link override Signal_Limit/_minval: Value=KOUTP_LFWhlRotDirTimeOut_flg_minval
      link override Signal_Override/_ovrdflg: Value=KOUTP_LFWhlRotDirTimeOut_flg_ovrdflg
      link override Signal_Override/_ovrdval: Value=KOUTP_LFWhlRotDirTimeOut_flg_ovrdval
  VAPM_LFWhlRotDir_enum_Inproc : FVT_lib/outp/OverrideAndLimit  SystemSampleTime=-1  VariantActivationTime=update diagram  Latency=0  AutoFrameSizeCalculation=off
      link override Signal_Limit/_maxval: Value=KOUTP_LFWhlRotDir_enum_maxval
      link override Signal_Limit/_minval: Value=KOUTP_LFWhlRotDir_enum_minval
      link override Signal_Override/_ovrdflg: Value=KOUTP_LFWhlRotDir_enum_ovrdflg
      link override Signal_Override/_ovrdval: Value=KOUTP_LFWhlRotDir_enum_ovrdval
  VAPM_LRPulseCountTimeOut_flg_Inproc : FVT_lib/outp/OverrideAndLimit  SystemSampleTime=-1  VariantActivationTime=update diagram  Latency=0  AutoFrameSizeCalculation=off
      link override Signal_Limit/_maxval: Value=KOUTP_LRPulseCountTimeOut_flg_maxval
      link override Signal_Limit/_minval: Value=KOUTP_LRPulseCountTimeOut_flg_minval
      link override Signal_Override/_ovrdflg: Value=KOUTP_LRPulseCountTimeOut_flg_ovrdflg
      link override Signal_Override/_ovrdval: Value=KOUTP_LRPulseCountTimeOut_flg_ovrdval
  VAPM_LRPulseCountVTimeOut_flg_Inproc : FVT_lib/outp/OverrideAndLimit  SystemSampleTime=-1  VariantActivationTime=update diagram  Latency=0  AutoFrameSizeCalculation=off
      link override Signal_Limit/_maxval: Value=KOUTP_LRPulseCountVTimeOut_flg_maxval
      link override Signal_Limit/_minval: Value=KOUTP_LRPulseCountVTimeOut_flg_minval
      link override Signal_Override/_ovrdflg: Value=KOUTP_LRPulseCountVTimeOut_flg_ovrdflg
      link override Signal_Override/_ovrdval: Value=KOUTP_LRPulseCountVTimeOut_flg_ovrdval
  VAPM_LRPulseCountV_flg_Inproc : FVT_lib/outp/OverrideAndLimit  SystemSampleTime=-1  VariantActivationTime=update diagram  Latency=0  AutoFrameSizeCalculation=off
      link override Signal_Limit/_maxval: Value=KOUTP_LRPulseCountV_flg_maxval
      link override Signal_Limit/_minval: Value=KOUTP_LRPulseCountV_flg_minval
      link override Signal_Override/_ovrdflg: Value=KOUTP_LRPulseCountV_flg_ovrdflg
      link override Signal_Override/_ovrdval: Value=KOUTP_LRPulseCountV_flg_ovrdval
  VAPM_LRPulseCount_enum_Inproc : FVT_lib/outp/OverrideAndLimit  SystemSampleTime=-1  VariantActivationTime=update diagram  Latency=0  AutoFrameSizeCalculation=off
      link override Signal_Limit/_maxval: Value=KOUTP_LRPulseCount_enum_maxval
      link override Signal_Limit/_minval: Value=KOUTP_LRPulseCount_enum_minval
      link override Signal_Override/_ovrdflg: Value=KOUTP_LRPulseCount_enum_ovrdflg
      link override Signal_Override/_ovrdval: Value=KOUTP_LRPulseCount_enum_ovrdval
  VAPM_LRRawWhlSpeedTimeOut_flg_Inproc : FVT_lib/outp/OverrideAndLimit  SystemSampleTime=-1  VariantActivationTime=update diagram  Latency=0  AutoFrameSizeCalculation=off
      link override Signal_Limit/_maxval: Value=KOUTP_LRRawWhlSpeedTimeOut_flg_maxval
      link override Signal_Limit/_minval: Value=KOUTP_LRRawWhlSpeedTimeOut_flg_minval
      link override Signal_Override/_ovrdflg: Value=KOUTP_LRRawWhlSpeedTimeOut_flg_ovrdflg
      link override Signal_Override/_ovrdval: Value=KOUTP_LRRawWhlSpeedTimeOut_flg_ovrdval
  VAPM_LRRawWhlSpeedVTimeOut_flg_Inproc : FVT_lib/outp/OverrideAndLimit  SystemSampleTime=-1  VariantActivationTime=update diagram  Latency=0  AutoFrameSizeCalculation=off
      link override Signal_Limit/_maxval: Value=KOUTP_LRRawWhlSpeedVTimeOut_flg_maxval
      link override Signal_Limit/_minval: Value=KOUTP_LRRawWhlSpeedVTimeOut_flg_minval
      link override Signal_Override/_ovrdflg: Value=KOUTP_LRRawWhlSpeedVTimeOut_flg_ovrdflg
      link override Signal_Override/_ovrdval: Value=KOUTP_LRRawWhlSpeedVTimeOut_flg_ovrdval
  VAPM_LRRawWhlSpeedV_flg_Inproc : FVT_lib/outp/OverrideAndLimit  SystemSampleTime=-1  VariantActivationTime=update diagram  Latency=0  AutoFrameSizeCalculation=off
      link override Signal_Limit/_maxval: Value=KOUTP_LRRawWhlSpeedV_flg_maxval
      link override Signal_Limit/_minval: Value=KOUTP_LRRawWhlSpeedV_flg_minval
      link override Signal_Override/_ovrdflg: Value=KOUTP_LRRawWhlSpeedV_flg_ovrdflg
      link override Signal_Override/_ovrdval: Value=KOUTP_LRRawWhlSpeedV_flg_ovrdval
  VAPM_LRRawWhlSpeed_kph_Inproc : FVT_lib/outp/OverrideAndLimit  SystemSampleTime=-1  VariantActivationTime=update diagram  Latency=0  AutoFrameSizeCalculation=off
      link override Signal_Limit/_maxval: Value=KOUTP_LRRawWhlSpeed_kph_maxval
      link override Signal_Limit/_minval: Value=KOUTP_LRRawWhlSpeed_kph_minval
      link override Signal_Override/_ovrdflg: Value=KOUTP_LRRawWhlSpeed_kph_ovrdflg
      link override Signal_Override/_ovrdval: Value=KOUTP_LRRawWhlSpeed_kph_ovrdval
  VAPM_LRWhlRotDirTimeOut_flg_Inproc : FVT_lib/outp/OverrideAndLimit  SystemSampleTime=-1  VariantActivationTime=update diagram  Latency=0  AutoFrameSizeCalculation=off
      link override Signal_Limit/_maxval: Value=KOUTP_LRWhlRotDirTimeOut_flg_maxval
      link override Signal_Limit/_minval: Value=KOUTP_LRWhlRotDirTimeOut_flg_minval
      link override Signal_Override/_ovrdflg: Value=KOUTP_LRWhlRotDirTimeOut_flg_ovrdflg
      link override Signal_Override/_ovrdval: Value=KOUTP_LRWhlRotDirTimeOut_flg_ovrdval
  VAPM_LRWhlRotDir_enum_Inproc : FVT_lib/outp/OverrideAndLimit  SystemSampleTime=-1  VariantActivationTime=update diagram  Latency=0  AutoFrameSizeCalculation=off
      link override Signal_Limit/_maxval: Value=KOUTP_LRWhlRotDir_enum_maxval
      link override Signal_Limit/_minval: Value=KOUTP_LRWhlRotDir_enum_minval
      link override Signal_Override/_ovrdflg: Value=KOUTP_LRWhlRotDir_enum_ovrdflg
      link override Signal_Override/_ovrdval: Value=KOUTP_LRWhlRotDir_enum_ovrdval
  VAPM_LatAccelTimeOut_flg_Inproc : FVT_lib/outp/OverrideAndLimit  SystemSampleTime=-1  VariantActivationTime=update diagram  Latency=0  AutoFrameSizeCalculation=off
      link override Signal_Limit/_maxval: Value=KOUTP_LatAccelTimeOut_flg_maxval
      link override Signal_Limit/_minval: Value=KOUTP_LatAccelTimeOut_flg_minval
      link override Signal_Override/_ovrdflg: Value=KOUTP_LatAccelTimeOut_flg_ovrdflg
      link override Signal_Override/_ovrdval: Value=KOUTP_LatAccelTimeOut_flg_ovrdval
  VAPM_LatAccelVTimeOut_flg_Inproc : FVT_lib/outp/OverrideAndLimit  SystemSampleTime=-1  VariantActivationTime=update diagram  Latency=0  AutoFrameSizeCalculation=off
      link override Signal_Limit/_maxval: Value=KOUTP_LatAccelVTimeOut_flg_maxval
      link override Signal_Limit/_minval: Value=KOUTP_LatAccelVTimeOut_flg_minval
      link override Signal_Override/_ovrdflg: Value=KOUTP_LatAccelVTimeOut_flg_ovrdflg
      link override Signal_Override/_ovrdval: Value=KOUTP_LatAccelVTimeOut_flg_ovrdval
  VAPM_LatAccelV_flg_Inproc : FVT_lib/outp/OverrideAndLimit  SystemSampleTime=-1  VariantActivationTime=update diagram  Latency=0  AutoFrameSizeCalculation=off
      link override Signal_Limit/_maxval: Value=KOUTP_LatAccelV_flg_maxval
      link override Signal_Limit/_minval: Value=KOUTP_LatAccelV_flg_minval
      link override Signal_Override/_ovrdflg: Value=KOUTP_LatAccelV_flg_ovrdflg
      link override Signal_Override/_ovrdval: Value=KOUTP_LatAccelV_flg_ovrdval
  VAPM_LatAccel_Gps_Inproc : FVT_lib/outp/OverrideAndLimit  SystemSampleTime=-1  VariantActivationTime=update diagram  Latency=0  AutoFrameSizeCalculation=off
      link override Signal_Limit/_maxval: Value=KOUTP_LatAccel_Gps_maxval
      link override Signal_Limit/_minval: Value=KOUTP_LatAccel_Gps_minval
      link override Signal_Override/_ovrdflg: Value=KOUTP_LatAccel_Gps_ovrdflg
      link override Signal_Override/_ovrdval: Value=KOUTP_LatAccel_Gps_ovrdval
  VAPM_LongAccelTimeOut_flg_Inproc : FVT_lib/outp/OverrideAndLimit  SystemSampleTime=-1  VariantActivationTime=update diagram  Latency=0  AutoFrameSizeCalculation=off
      link override Signal_Limit/_maxval: Value=KOUTP_LongAccelTimeOut_flg_maxval
      link override Signal_Limit/_minval: Value=KOUTP_LongAccelTimeOut_flg_minval
      link override Signal_Override/_ovrdflg: Value=KOUTP_LongAccelTimeOut_flg_ovrdflg
      link override Signal_Override/_ovrdval: Value=KOUTP_LongAccelTimeOut_flg_ovrdval
  VAPM_LongAccelVTimeOut_flg_Inproc : FVT_lib/outp/OverrideAndLimit  SystemSampleTime=-1  VariantActivationTime=update diagram  Latency=0  AutoFrameSizeCalculation=off
      link override Signal_Limit/_maxval: Value=KOUTP_LongAccelVTimeOut_flg_maxval
      link override Signal_Limit/_minval: Value=KOUTP_LongAccelVTimeOut_flg_minval
      link override Signal_Override/_ovrdflg: Value=KOUTP_LongAccelVTimeOut_flg_ovrdflg
      link override Signal_Override/_ovrdval: Value=KOUTP_LongAccelVTimeOut_flg_ovrdval
  VAPM_LongAccelV_flg_Inproc : FVT_lib/outp/OverrideAndLimit  SystemSampleTime=-1  VariantActivationTime=update diagram  Latency=0  AutoFrameSizeCalculation=off
      link override Signal_Limit/_maxval: Value=KOUTP_LongAccelV_flg_maxval
      link override Signal_Limit/_minval: Value=KOUTP_LongAccelV_flg_minval
      link override Signal_Override/_ovrdflg: Value=KOUTP_LongAccelV_flg_ovrdflg
      link override Signal_Override/_ovrdval: Value=KOUTP_LongAccelV_flg_ovrdval
  VAPM_LongAccel_Gps_Inproc : FVT_lib/outp/OverrideAndLimit  SystemSampleTime=-1  VariantActivationTime=update diagram  Latency=0  AutoFrameSizeCalculation=off
      link override Signal_Limit/_maxval: Value=KOUTP_LongAccel_Gps_maxval
      link override Signal_Limit/_minval: Value=KOUTP_LongAccel_Gps_minval
      link override Signal_Override/_ovrdflg: Value=KOUTP_LongAccel_Gps_ovrdflg
      link override Signal_Override/_ovrdval: Value=KOUTP_LongAccel_Gps_ovrdval
  VAPM_MCPressureTimeOut_flg_Inproc : FVT_lib/outp/OverrideAndLimit  SystemSampleTime=-1  VariantActivationTime=update diagram  Latency=0  AutoFrameSizeCalculation=off
      link override Signal_Limit/_maxval: Value=KOUTP_MCPressureTimeOut_flg_maxval
      link override Signal_Limit/_minval: Value=KOUTP_MCPressureTimeOut_flg_minval
      link override Signal_Override/_ovrdflg: Value=KOUTP_MCPressureTimeOut_flg_ovrdflg
      link override Signal_Override/_ovrdval: Value=KOUTP_MCPressureTimeOut_flg_ovrdval
  VAPM_MCPressureVTimeOut_flg_Inproc : FVT_lib/outp/OverrideAndLimit  SystemSampleTime=-1  VariantActivationTime=update diagram  Latency=0  AutoFrameSizeCalculation=off
      link override Signal_Limit/_maxval: Value=KOUTP_MCPressureVTimeOut_flg_maxval
      link override Signal_Limit/_minval: Value=KOUTP_MCPressureVTimeOut_flg_minval
      link override Signal_Override/_ovrdflg: Value=KOUTP_MCPressureVTimeOut_flg_ovrdflg
      link override Signal_Override/_ovrdval: Value=KOUTP_MCPressureVTimeOut_flg_ovrdval
  VAPM_MCPressureV_bar_Inproc : FVT_lib/outp/OverrideAndLimit  SystemSampleTime=-1  VariantActivationTime=update diagram  Latency=0  AutoFrameSizeCalculation=off
      link override Signal_Limit/_maxval: Value=KOUTP_MCPressureV_bar_maxval
      link override Signal_Limit/_minval: Value=KOUTP_MCPressureV_bar_minval
      link override Signal_Override/_ovrdflg: Value=KOUTP_MCPressureV_bar_ovrdflg
      link override Signal_Override/_ovrdval: Value=KOUTP_MCPressureV_bar_ovrdval
  VAPM_MCPressure_bar_Inproc : FVT_lib/outp/OverrideAndLimit  SystemSampleTime=-1  VariantActivationTime=update diagram  Latency=0  AutoFrameSizeCalculation=off
      link override Signal_Limit/_maxval: Value=KOUTP_MCPressure_bar_maxval
      link override Signal_Limit/_minval: Value=KOUTP_MCPressure_bar_minval
      link override Signal_Override/_ovrdflg: Value=KOUTP_MCPressure_bar_ovrdflg
      link override Signal_Override/_ovrdval: Value=KOUTP_MCPressure_bar_ovrdval
  VAPM_ModOperation_enum_Inproc : FVT_lib/outp/OverrideAndLimit  SystemSampleTime=-1  VariantActivationTime=update diagram  Latency=0  AutoFrameSizeCalculation=off
      link override Signal_Limit/_maxval: Value=KOUTP_ModOperation_enum_maxval
      link override Signal_Limit/_minval: Value=KOUTP_ModOperation_enum_minval
      link override Signal_Override/_ovrdflg: Value=KOUTP_ModOperation_enum_ovrdflg
      link override Signal_Override/_ovrdval: Value=KOUTP_ModOperation_enum_ovrdval
  VAPM_PASAFCL_enum_Inproc : FVT_lib/outp/OverrideAndLimit  SystemSampleTime=-1  VariantActivationTime=update diagram  Latency=0  AutoFrameSizeCalculation=off
      link override Signal_Limit/_maxval: Value=KOUTP_PASAFCL_enum_maxval
      link override Signal_Limit/_minval: Value=KOUTP_PASAFCL_enum_minval
      link override Signal_Override/_ovrdflg: Value=KOUTP_PASAFCL_enum_ovrdflg
      link override Signal_Override/_ovrdval: Value=KOUTP_PASAFCL_enum_ovrdval
  VAPM_PASAFCR_enum_Inproc : FVT_lib/outp/OverrideAndLimit  SystemSampleTime=-1  VariantActivationTime=update diagram  Latency=0  AutoFrameSizeCalculation=off
      link override Signal_Limit/_maxval: Value=KOUTP_PASAFCR_enum_maxval
      link override Signal_Limit/_minval: Value=KOUTP_PASAFCR_enum_minval
      link override Signal_Override/_ovrdflg: Value=KOUTP_PASAFCR_enum_ovrdflg
      link override Signal_Override/_ovrdval: Value=KOUTP_PASAFCR_enum_ovrdval
  VAPM_PASAFML_enum_Inproc : FVT_lib/outp/OverrideAndLimit  SystemSampleTime=-1  VariantActivationTime=update diagram  Latency=0  AutoFrameSizeCalculation=off
      link override Signal_Limit/_maxval: Value=KOUTP_PASAFML_enum_maxval
      link override Signal_Limit/_minval: Value=KOUTP_PASAFML_enum_minval
      link override Signal_Override/_ovrdflg: Value=KOUTP_PASAFML_enum_ovrdflg
      link override Signal_Override/_ovrdval: Value=KOUTP_PASAFML_enum_ovrdval
  VAPM_PASAFMR_enum_Inproc : FVT_lib/outp/OverrideAndLimit  SystemSampleTime=-1  VariantActivationTime=update diagram  Latency=0  AutoFrameSizeCalculation=off
      link override Signal_Limit/_maxval: Value=KOUTP_PASAFMR_enum_maxval
      link override Signal_Limit/_minval: Value=KOUTP_PASAFMR_enum_minval
      link override Signal_Override/_ovrdflg: Value=KOUTP_PASAFMR_enum_ovrdflg
      link override Signal_Override/_ovrdval: Value=KOUTP_PASAFMR_enum_ovrdval
  VAPM_PASARCL_enum_Inproc : FVT_lib/outp/OverrideAndLimit  SystemSampleTime=-1  VariantActivationTime=update diagram  Latency=0  AutoFrameSizeCalculation=off
      link override Signal_Limit/_maxval: Value=KOUTP_PASARCL_enum_maxval
      link override Signal_Limit/_minval: Value=KOUTP_PASARCL_enum_minval
      link override Signal_Override/_ovrdflg: Value=KOUTP_PASARCL_enum_ovrdflg
      link override Signal_Override/_ovrdval: Value=KOUTP_PASARCL_enum_ovrdval
  VAPM_PASARCR_enum_Inproc : FVT_lib/outp/OverrideAndLimit  SystemSampleTime=-1  VariantActivationTime=update diagram  Latency=0  AutoFrameSizeCalculation=off
      link override Signal_Limit/_maxval: Value=KOUTP_PASARCR_enum_maxval
      link override Signal_Limit/_minval: Value=KOUTP_PASARCR_enum_minval
      link override Signal_Override/_ovrdflg: Value=KOUTP_PASARCR_enum_ovrdflg
      link override Signal_Override/_ovrdval: Value=KOUTP_PASARCR_enum_ovrdval
  VAPM_PASARML_enum_Inproc : FVT_lib/outp/OverrideAndLimit  SystemSampleTime=-1  VariantActivationTime=update diagram  Latency=0  AutoFrameSizeCalculation=off
      link override Signal_Limit/_maxval: Value=KOUTP_PASARML_enum_maxval
      link override Signal_Limit/_minval: Value=KOUTP_PASARML_enum_minval
      link override Signal_Override/_ovrdflg: Value=KOUTP_PASARML_enum_ovrdflg
      link override Signal_Override/_ovrdval: Value=KOUTP_PASARML_enum_ovrdval
  VAPM_PASARMR_enum_Inproc : FVT_lib/outp/OverrideAndLimit  SystemSampleTime=-1  VariantActivationTime=update diagram  Latency=0  AutoFrameSizeCalculation=off
      link override Signal_Limit/_maxval: Value=KOUTP_PASARMR_enum_maxval
      link override Signal_Limit/_minval: Value=KOUTP_PASARMR_enum_minval
      link override Signal_Override/_ovrdflg: Value=KOUTP_PASARMR_enum_ovrdflg
      link override Signal_Override/_ovrdval: Value=KOUTP_PASARMR_enum_ovrdval
  VAPM_PASDFCL_cm_Inproc : FVT_lib/outp/OverrideAndLimit  SystemSampleTime=-1  VariantActivationTime=update diagram  Latency=0  AutoFrameSizeCalculation=off
      link override Signal_Limit/_maxval: Value=KOUTP_PASDFCL_cm_maxval
      link override Signal_Limit/_minval: Value=KOUTP_PASDFCL_cm_minval
      link override Signal_Override/_ovrdflg: Value=KOUTP_PASDFCL_cm_ovrdflg
      link override Signal_Override/_ovrdval: Value=KOUTP_PASDFCL_cm_ovrdval
  VAPM_PASDFCR_cm_Inproc : FVT_lib/outp/OverrideAndLimit  SystemSampleTime=-1  VariantActivationTime=update diagram  Latency=0  AutoFrameSizeCalculation=off
      link override Signal_Limit/_maxval: Value=KOUTP_PASDFCR_cm_maxval
      link override Signal_Limit/_minval: Value=KOUTP_PASDFCR_cm_minval
      link override Signal_Override/_ovrdflg: Value=KOUTP_PASDFCR_cm_ovrdflg
      link override Signal_Override/_ovrdval: Value=KOUTP_PASDFCR_cm_ovrdval
  VAPM_PASDFML_cm_Inproc : FVT_lib/outp/OverrideAndLimit  SystemSampleTime=-1  VariantActivationTime=update diagram  Latency=0  AutoFrameSizeCalculation=off
      link override Signal_Limit/_maxval: Value=KOUTP_PASDFML_cm_maxval
      link override Signal_Limit/_minval: Value=KOUTP_PASDFML_cm_minval
      link override Signal_Override/_ovrdflg: Value=KOUTP_PASDFML_cm_ovrdflg
      link override Signal_Override/_ovrdval: Value=KOUTP_PASDFML_cm_ovrdval
  VAPM_PASDFMR_cm_Inproc : FVT_lib/outp/OverrideAndLimit  SystemSampleTime=-1  VariantActivationTime=update diagram  Latency=0  AutoFrameSizeCalculation=off
      link override Signal_Limit/_maxval: Value=KOUTP_PASDFMR_cm_maxval
      link override Signal_Limit/_minval: Value=KOUTP_PASDFMR_cm_minval
      link override Signal_Override/_ovrdflg: Value=KOUTP_PASDFMR_cm_ovrdflg
      link override Signal_Override/_ovrdval: Value=KOUTP_PASDFMR_cm_ovrdval
  VAPM_PASDRCL_cm_Inproc : FVT_lib/outp/OverrideAndLimit  SystemSampleTime=-1  VariantActivationTime=update diagram  Latency=0  AutoFrameSizeCalculation=off
      link override Signal_Limit/_maxval: Value=KOUTP_PASDRCL_cm_maxval
      link override Signal_Limit/_minval: Value=KOUTP_PASDRCL_cm_minval
      link override Signal_Override/_ovrdflg: Value=KOUTP_PASDRCL_cm_ovrdflg
      link override Signal_Override/_ovrdval: Value=KOUTP_PASDRCL_cm_ovrdval
  VAPM_PASDRCR_cm_Inproc : FVT_lib/outp/OverrideAndLimit  SystemSampleTime=-1  VariantActivationTime=update diagram  Latency=0  AutoFrameSizeCalculation=off
      link override Signal_Limit/_maxval: Value=KOUTP_PASDRCR_cm_maxval
      link override Signal_Limit/_minval: Value=KOUTP_PASDRCR_cm_minval
      link override Signal_Override/_ovrdflg: Value=KOUTP_PASDRCR_cm_ovrdflg
      link override Signal_Override/_ovrdval: Value=KOUTP_PASDRCR_cm_ovrdval
  VAPM_PASDRML_cm_Inproc : FVT_lib/outp/OverrideAndLimit  SystemSampleTime=-1  VariantActivationTime=update diagram  Latency=0  AutoFrameSizeCalculation=off
      link override Signal_Limit/_maxval: Value=KOUTP_PASDRML_cm_maxval
      link override Signal_Limit/_minval: Value=KOUTP_PASDRML_cm_minval
      link override Signal_Override/_ovrdflg: Value=KOUTP_PASDRML_cm_ovrdflg
      link override Signal_Override/_ovrdval: Value=KOUTP_PASDRML_cm_ovrdval
  VAPM_PASDRMR_cm_Inproc : FVT_lib/outp/OverrideAndLimit  SystemSampleTime=-1  VariantActivationTime=update diagram  Latency=0  AutoFrameSizeCalculation=off
      link override Signal_Limit/_maxval: Value=KOUTP_PASDRMR_cm_maxval
      link override Signal_Limit/_minval: Value=KOUTP_PASDRMR_cm_minval
      link override Signal_Override/_ovrdflg: Value=KOUTP_PASDRMR_cm_ovrdflg
      link override Signal_Override/_ovrdval: Value=KOUTP_PASDRMR_cm_ovrdval
  VAPM_RFPulseCountTimeOut_flg_Inproc : FVT_lib/outp/OverrideAndLimit  SystemSampleTime=-1  VariantActivationTime=update diagram  Latency=0  AutoFrameSizeCalculation=off
      link override Signal_Limit/_maxval: Value=KOUTP_RFPulseCountTimeOut_flg_maxval
      link override Signal_Limit/_minval: Value=KOUTP_RFPulseCountTimeOut_flg_minval
      link override Signal_Override/_ovrdflg: Value=KOUTP_RFPulseCountTimeOut_flg_ovrdflg
      link override Signal_Override/_ovrdval: Value=KOUTP_RFPulseCountTimeOut_flg_ovrdval
  VAPM_RFPulseCountVTimeOut_flg_Inproc : FVT_lib/outp/OverrideAndLimit  SystemSampleTime=-1  VariantActivationTime=update diagram  Latency=0  AutoFrameSizeCalculation=off
      link override Signal_Limit/_maxval: Value=KOUTP_RFPulseCountVTimeOut_flg_maxval
      link override Signal_Limit/_minval: Value=KOUTP_RFPulseCountVTimeOut_flg_minval
      link override Signal_Override/_ovrdflg: Value=KOUTP_RFPulseCountVTimeOut_flg_ovrdflg
      link override Signal_Override/_ovrdval: Value=KOUTP_RFPulseCountVTimeOut_flg_ovrdval
  VAPM_RFPulseCountV_flg_Inproc : FVT_lib/outp/OverrideAndLimit  SystemSampleTime=-1  VariantActivationTime=update diagram  Latency=0  AutoFrameSizeCalculation=off
      link override Signal_Limit/_maxval: Value=KOUTP_RFPulseCountV_flg_maxval
      link override Signal_Limit/_minval: Value=KOUTP_RFPulseCountV_flg_minval
      link override Signal_Override/_ovrdflg: Value=KOUTP_RFPulseCountV_flg_ovrdflg
      link override Signal_Override/_ovrdval: Value=KOUTP_RFPulseCountV_flg_ovrdval
  VAPM_RFPulseCount_enum_Inproc : FVT_lib/outp/OverrideAndLimit  SystemSampleTime=-1  VariantActivationTime=update diagram  Latency=0  AutoFrameSizeCalculation=off
      link override Signal_Limit/_maxval: Value=KOUTP_RFPulseCount_enum_maxval
      link override Signal_Limit/_minval: Value=KOUTP_RFPulseCount_enum_minval
      link override Signal_Override/_ovrdflg: Value=KOUTP_RFPulseCount_enum_ovrdflg
      link override Signal_Override/_ovrdval: Value=KOUTP_RFPulseCount_enum_ovrdval
  VAPM_RFRawWhlSpeedTimeOut_flg_Inproc : FVT_lib/outp/OverrideAndLimit  SystemSampleTime=-1  VariantActivationTime=update diagram  Latency=0  AutoFrameSizeCalculation=off
      link override Signal_Limit/_maxval: Value=KOUTP_RFRawWhlSpeedTimeOut_flg_maxval
      link override Signal_Limit/_minval: Value=KOUTP_RFRawWhlSpeedTimeOut_flg_minval
      link override Signal_Override/_ovrdflg: Value=KOUTP_RFRawWhlSpeedTimeOut_flg_ovrdflg
      link override Signal_Override/_ovrdval: Value=KOUTP_RFRawWhlSpeedTimeOut_flg_ovrdval
  VAPM_RFRawWhlSpeedVTimeOut_flg_Inproc : FVT_lib/outp/OverrideAndLimit  SystemSampleTime=-1  VariantActivationTime=update diagram  Latency=0  AutoFrameSizeCalculation=off
      link override Signal_Limit/_maxval: Value=KOUTP_RFRawWhlSpeedVTimeOut_flg_maxval
      link override Signal_Limit/_minval: Value=KOUTP_RFRawWhlSpeedVTimeOut_flg_minval
      link override Signal_Override/_ovrdflg: Value=KOUTP_RFRawWhlSpeedVTimeOut_flg_ovrdflg
      link override Signal_Override/_ovrdval: Value=KOUTP_RFRawWhlSpeedVTimeOut_flg_ovrdval
  VAPM_RFRawWhlSpeedV_flg_Inproc : FVT_lib/outp/OverrideAndLimit  SystemSampleTime=-1  VariantActivationTime=update diagram  Latency=0  AutoFrameSizeCalculation=off
      link override Signal_Limit/_maxval: Value=KOUTP_RFRawWhlSpeedV_flg_maxval
      link override Signal_Limit/_minval: Value=KOUTP_RFRawWhlSpeedV_flg_minval
      link override Signal_Override/_ovrdflg: Value=KOUTP_RFRawWhlSpeedV_flg_ovrdflg
      link override Signal_Override/_ovrdval: Value=KOUTP_RFRawWhlSpeedV_flg_ovrdval
  VAPM_RFRawWhlSpeed_kph_Inproc : FVT_lib/outp/OverrideAndLimit  SystemSampleTime=-1  VariantActivationTime=update diagram  Latency=0  AutoFrameSizeCalculation=off
      link override Signal_Limit/_maxval: Value=KOUTP_RFRawWhlSpeed_kph_maxval
      link override Signal_Limit/_minval: Value=KOUTP_RFRawWhlSpeed_kph_minval
      link override Signal_Override/_ovrdflg: Value=KOUTP_RFRawWhlSpeed_kph_ovrdflg
      link override Signal_Override/_ovrdval: Value=KOUTP_RFRawWhlSpeed_kph_ovrdval
  VAPM_RFWhlRotDirTimeOut_flg_Inproc : FVT_lib/outp/OverrideAndLimit  SystemSampleTime=-1  VariantActivationTime=update diagram  Latency=0  AutoFrameSizeCalculation=off
      link override Signal_Limit/_maxval: Value=KOUTP_RFWhlRotDirTimeOut_flg_maxval
      link override Signal_Limit/_minval: Value=KOUTP_RFWhlRotDirTimeOut_flg_minval
      link override Signal_Override/_ovrdflg: Value=KOUTP_RFWhlRotDirTimeOut_flg_ovrdflg
      link override Signal_Override/_ovrdval: Value=KOUTP_RFWhlRotDirTimeOut_flg_ovrdval
  VAPM_RFWhlRotDir_enum_Inproc : FVT_lib/outp/OverrideAndLimit  SystemSampleTime=-1  VariantActivationTime=update diagram  Latency=0  AutoFrameSizeCalculation=off
      link override Signal_Limit/_maxval: Value=KOUTP_RFWhlRotDir_enum_maxval
      link override Signal_Limit/_minval: Value=KOUTP_RFWhlRotDir_enum_minval
      link override Signal_Override/_ovrdflg: Value=KOUTP_RFWhlRotDir_enum_ovrdflg
      link override Signal_Override/_ovrdval: Value=KOUTP_RFWhlRotDir_enum_ovrdval
  VAPM_RRPulseCountTimeOut_flg_Inproc : FVT_lib/outp/OverrideAndLimit  SystemSampleTime=-1  VariantActivationTime=update diagram  Latency=0  AutoFrameSizeCalculation=off
      link override Signal_Limit/_maxval: Value=KOUTP_RRPulseCountTimeOut_flg_maxval
      link override Signal_Limit/_minval: Value=KOUTP_RRPulseCountTimeOut_flg_minval
      link override Signal_Override/_ovrdflg: Value=KOUTP_RRPulseCountTimeOut_flg_ovrdflg
      link override Signal_Override/_ovrdval: Value=KOUTP_RRPulseCountTimeOut_flg_ovrdval
  VAPM_RRPulseCountVTimeOut_flg_Inproc : FVT_lib/outp/OverrideAndLimit  SystemSampleTime=-1  VariantActivationTime=update diagram  Latency=0  AutoFrameSizeCalculation=off
      link override Signal_Limit/_maxval: Value=KOUTP_RRPulseCountVTimeOut_flg_maxval
      link override Signal_Limit/_minval: Value=KOUTP_RRPulseCountVTimeOut_flg_minval
      link override Signal_Override/_ovrdflg: Value=KOUTP_RRPulseCountVTimeOut_flg_ovrdflg
      link override Signal_Override/_ovrdval: Value=KOUTP_RRPulseCountVTimeOut_flg_ovrdval
  VAPM_RRPulseCountV_flg_Inproc : FVT_lib/outp/OverrideAndLimit  SystemSampleTime=-1  VariantActivationTime=update diagram  Latency=0  AutoFrameSizeCalculation=off
      link override Signal_Limit/_maxval: Value=KOUTP_RRPulseCountV_flg_maxval
      link override Signal_Limit/_minval: Value=KOUTP_RRPulseCountV_flg_minval
      link override Signal_Override/_ovrdflg: Value=KOUTP_RRPulseCountV_flg_ovrdflg
      link override Signal_Override/_ovrdval: Value=KOUTP_RRPulseCountV_flg_ovrdval
  VAPM_RRPulseCount_enum_Inproc : FVT_lib/outp/OverrideAndLimit  SystemSampleTime=-1  VariantActivationTime=update diagram  Latency=0  AutoFrameSizeCalculation=off
      link override Signal_Limit/_maxval: Value=KOUTP_RRPulseCount_enum_maxval
      link override Signal_Limit/_minval: Value=KOUTP_RRPulseCount_enum_minval
      link override Signal_Override/_ovrdflg: Value=KOUTP_RRPulseCount_enum_ovrdflg
      link override Signal_Override/_ovrdval: Value=KOUTP_RRPulseCount_enum_ovrdval
  VAPM_RRRawWhlSpeedTimeOut_flg_Inproc : FVT_lib/outp/OverrideAndLimit  SystemSampleTime=-1  VariantActivationTime=update diagram  Latency=0  AutoFrameSizeCalculation=off
      link override Signal_Limit/_maxval: Value=KOUTP_RRRawWhlSpeedTimeOut_flg_maxval
      link override Signal_Limit/_minval: Value=KOUTP_RRRawWhlSpeedTimeOut_flg_minval
      link override Signal_Override/_ovrdflg: Value=KOUTP_RRRawWhlSpeedTimeOut_flg_ovrdflg
      link override Signal_Override/_ovrdval: Value=KOUTP_RRRawWhlSpeedTimeOut_flg_ovrdval
  VAPM_RRRawWhlSpeedVTimeOut_flg_Inproc : FVT_lib/outp/OverrideAndLimit  SystemSampleTime=-1  VariantActivationTime=update diagram  Latency=0  AutoFrameSizeCalculation=off
      link override Signal_Limit/_maxval: Value=KOUTP_RRRawWhlSpeedVTimeOut_flg_maxval
      link override Signal_Limit/_minval: Value=KOUTP_RRRawWhlSpeedVTimeOut_flg_minval
      link override Signal_Override/_ovrdflg: Value=KOUTP_RRRawWhlSpeedVTimeOut_flg_ovrdflg
      link override Signal_Override/_ovrdval: Value=KOUTP_RRRawWhlSpeedVTimeOut_flg_ovrdval
  VAPM_RRRawWhlSpeedV_flg_Inproc : FVT_lib/outp/OverrideAndLimit  SystemSampleTime=-1  VariantActivationTime=update diagram  Latency=0  AutoFrameSizeCalculation=off
      link override Signal_Limit/_maxval: Value=KOUTP_RRRawWhlSpeedV_flg_maxval
      link override Signal_Limit/_minval: Value=KOUTP_RRRawWhlSpeedV_flg_minval
      link override Signal_Override/_ovrdflg: Value=KOUTP_RRRawWhlSpeedV_flg_ovrdflg
      link override Signal_Override/_ovrdval: Value=KOUTP_RRRawWhlSpeedV_flg_ovrdval
  VAPM_RRRawWhlSpeed_kph_Inproc : FVT_lib/outp/OverrideAndLimit  SystemSampleTime=-1  VariantActivationTime=update diagram  Latency=0  AutoFrameSizeCalculation=off
      link override Signal_Limit/_maxval: Value=KOUTP_RRRawWhlSpeed_kph_maxval
      link override Signal_Limit/_minval: Value=KOUTP_RRRawWhlSpeed_kph_minval
      link override Signal_Override/_ovrdflg: Value=KOUTP_RRRawWhlSpeed_kph_ovrdflg
      link override Signal_Override/_ovrdval: Value=KOUTP_RRRawWhlSpeed_kph_ovrdval
  VAPM_RRWhlRotDirTimeOut_flg_Inproc : FVT_lib/outp/OverrideAndLimit  SystemSampleTime=-1  VariantActivationTime=update diagram  Latency=0  AutoFrameSizeCalculation=off
      link override Signal_Limit/_maxval: Value=KOUTP_RRWhlRotDirTimeOut_flg_maxval
      link override Signal_Limit/_minval: Value=KOUTP_RRWhlRotDirTimeOut_flg_minval
      link override Signal_Override/_ovrdflg: Value=KOUTP_RRWhlRotDirTimeOut_flg_ovrdflg
      link override Signal_Override/_ovrdval: Value=KOUTP_RRWhlRotDirTimeOut_flg_ovrdval
  VAPM_RRWhlRotDir_enum_Inproc : FVT_lib/outp/OverrideAndLimit  SystemSampleTime=-1  VariantActivationTime=update diagram  Latency=0  AutoFrameSizeCalculation=off
      link override Signal_Limit/_maxval: Value=KOUTP_RRWhlRotDir_enum_maxval
      link override Signal_Limit/_minval: Value=KOUTP_RRWhlRotDir_enum_minval
      link override Signal_Override/_ovrdflg: Value=KOUTP_RRWhlRotDir_enum_ovrdflg
      link override Signal_Override/_ovrdval: Value=KOUTP_RRWhlRotDir_enum_ovrdval
  VAPM_SASAngleTimeOut_flg_Inproc : FVT_lib/outp/OverrideAndLimit  SystemSampleTime=-1  VariantActivationTime=update diagram  Latency=0  AutoFrameSizeCalculation=off
      link override Signal_Limit/_maxval: Value=KOUTP_SASAngleTimeOut_flg_maxval
      link override Signal_Limit/_minval: Value=KOUTP_SASAngleTimeOut_flg_minval
      link override Signal_Override/_ovrdflg: Value=KOUTP_SASAngleTimeOut_flg_ovrdflg
      link override Signal_Override/_ovrdval: Value=KOUTP_SASAngleTimeOut_flg_ovrdval
  VAPM_SASAngle_Deg_Inproc : FVT_lib/outp/OverrideAndLimit  SystemSampleTime=-1  VariantActivationTime=update diagram  Latency=0  AutoFrameSizeCalculation=off
      link override Signal_Limit/_maxval: Value=KOUTP_SASAngle_Deg_maxval
      link override Signal_Limit/_minval: Value=KOUTP_SASAngle_Deg_minval
      link override Signal_Override/_ovrdflg: Value=KOUTP_SASAngle_Deg_ovrdflg
      link override Signal_Override/_ovrdval: Value=KOUTP_SASAngle_Deg_ovrdval
  VAPM_SASCALTimeOut_flg_Inproc : FVT_lib/outp/OverrideAndLimit  SystemSampleTime=-1  VariantActivationTime=update diagram  Latency=0  AutoFrameSizeCalculation=off
      link override Signal_Limit/_maxval: Value=KOUTP_SASCALTimeOut_flg_maxval
      link override Signal_Limit/_minval: Value=KOUTP_SASCALTimeOut_flg_minval
      link override Signal_Override/_ovrdflg: Value=KOUTP_SASCALTimeOut_flg_ovrdflg
      link override Signal_Override/_ovrdval: Value=KOUTP_SASCALTimeOut_flg_ovrdval
  VAPM_SASCAL_flg_Inproc : FVT_lib/outp/OverrideAndLimit  SystemSampleTime=-1  VariantActivationTime=update diagram  Latency=0  AutoFrameSizeCalculation=off
      link override Signal_Limit/_maxval: Value=KOUTP_SASCAL_flg_maxval
      link override Signal_Limit/_minval: Value=KOUTP_SASCAL_flg_minval
      link override Signal_Override/_ovrdflg: Value=KOUTP_SASCAL_flg_ovrdflg
      link override Signal_Override/_ovrdval: Value=KOUTP_SASCAL_flg_ovrdval
  VAPM_SASSpeedTimeOut_flg_Inproc : FVT_lib/outp/OverrideAndLimit  SystemSampleTime=-1  VariantActivationTime=update diagram  Latency=0  AutoFrameSizeCalculation=off
      link override Signal_Limit/_maxval: Value=KOUTP_SASSpeedTimeOut_flg_maxval
      link override Signal_Limit/_minval: Value=KOUTP_SASSpeedTimeOut_flg_minval
      link override Signal_Override/_ovrdflg: Value=KOUTP_SASSpeedTimeOut_flg_ovrdflg
      link override Signal_Override/_ovrdval: Value=KOUTP_SASSpeedTimeOut_flg_ovrdval
  VAPM_SASSpeedValidTimeOut_flg_Inproc : FVT_lib/outp/OverrideAndLimit  SystemSampleTime=-1  VariantActivationTime=update diagram  Latency=0  AutoFrameSizeCalculation=off
      link override Signal_Limit/_maxval: Value=KOUTP_SASSpeedValidTimeOut_flg_maxval
      link override Signal_Limit/_minval: Value=KOUTP_SASSpeedValidTimeOut_flg_minval
      link override Signal_Override/_ovrdflg: Value=KOUTP_SASSpeedValidTimeOut_flg_ovrdflg
      link override Signal_Override/_ovrdval: Value=KOUTP_SASSpeedValidTimeOut_flg_ovrdval
  VAPM_SASSpeedValid_flg_Inproc : FVT_lib/outp/OverrideAndLimit  SystemSampleTime=-1  VariantActivationTime=update diagram  Latency=0  AutoFrameSizeCalculation=off
      link override Signal_Limit/_maxval: Value=KOUTP_SASSpeedValid_flg_maxval
      link override Signal_Limit/_minval: Value=KOUTP_SASSpeedValid_flg_minval
      link override Signal_Override/_ovrdflg: Value=KOUTP_SASSpeedValid_flg_ovrdflg
      link override Signal_Override/_ovrdval: Value=KOUTP_SASSpeedValid_flg_ovrdval
  VAPM_SASSpeed_degps_Inproc : FVT_lib/outp/OverrideAndLimit  SystemSampleTime=-1  VariantActivationTime=update diagram  Latency=0  AutoFrameSizeCalculation=off
      link override Signal_Limit/_maxval: Value=KOUTP_SASSpeed_degps_maxval
      link override Signal_Limit/_minval: Value=KOUTP_SASSpeed_degps_minval
      link override Signal_Override/_ovrdflg: Value=KOUTP_SASSpeed_degps_ovrdflg
      link override Signal_Override/_ovrdval: Value=KOUTP_SASSpeed_degps_ovrdval
  VAPM_SASVTimeOut_flg_Inproc : FVT_lib/outp/OverrideAndLimit  SystemSampleTime=-1  VariantActivationTime=update diagram  Latency=0  AutoFrameSizeCalculation=off
      link override Signal_Limit/_maxval: Value=KOUTP_SASVTimeOut_flg_maxval
      link override Signal_Limit/_minval: Value=KOUTP_SASVTimeOut_flg_minval
      link override Signal_Override/_ovrdflg: Value=KOUTP_SASVTimeOut_flg_ovrdflg
      link override Signal_Override/_ovrdval: Value=KOUTP_SASVTimeOut_flg_ovrdval
  VAPM_SASV_flg_Inproc : FVT_lib/outp/OverrideAndLimit  SystemSampleTime=-1  VariantActivationTime=update diagram  Latency=0  AutoFrameSizeCalculation=off
      link override Signal_Limit/_maxval: Value=KOUTP_SASV_flg_maxval
      link override Signal_Limit/_minval: Value=KOUTP_SASV_flg_minval
      link override Signal_Override/_ovrdflg: Value=KOUTP_SASV_flg_ovrdflg
      link override Signal_Override/_ovrdval: Value=KOUTP_SASV_flg_ovrdval
  VAPM_SNSRLayout_enum_Inproc : FVT_lib/outp/OverrideAndLimit  SystemSampleTime=-1  VariantActivationTime=update diagram  Latency=0  AutoFrameSizeCalculation=off
      link override Signal_Limit/_maxval: Value=KOUTP_SNSRLayout_enum_maxval
      link override Signal_Limit/_minval: Value=KOUTP_SNSRLayout_enum_minval
      link override Signal_Override/_ovrdflg: Value=KOUTP_SNSRLayout_enum_ovrdflg
      link override Signal_Override/_ovrdval: Value=KOUTP_SNSRLayout_enum_ovrdval
  VAPM_ShifterHandleCmdTimeOut_flg_Inproc : FVT_lib/outp/OverrideAndLimit  SystemSampleTime=-1  VariantActivationTime=update diagram  Latency=0  AutoFrameSizeCalculation=off
      link override Signal_Limit/_maxval: Value=KOUTP_ShifterHandleCmdTimeOut_flg_maxval
      link override Signal_Limit/_minval: Value=KOUTP_ShifterHandleCmdTimeOut_flg_minval
      link override Signal_Override/_ovrdflg: Value=KOUTP_ShifterHandleCmdTimeOut_flg_ovrdflg
      link override Signal_Override/_ovrdval: Value=KOUTP_ShifterHandleCmdTimeOut_flg_ovrdval
  VAPM_ShifterHandleCmd_enum_Inproc : FVT_lib/outp/OverrideAndLimit  SystemSampleTime=-1  VariantActivationTime=update diagram  Latency=0  AutoFrameSizeCalculation=off
      link override Signal_Limit/_maxval: Value=KOUTP_ShifterHandleCmd_enum_maxval
      link override Signal_Limit/_minval: Value=KOUTP_ShifterHandleCmd_enum_minval
      link override Signal_Override/_ovrdflg: Value=KOUTP_ShifterHandleCmd_enum_ovrdflg
      link override Signal_Override/_ovrdval: Value=KOUTP_ShifterHandleCmd_enum_ovrdval
  VAPM_StaFSya_flg_Inproc : FVT_lib/outp/OverrideAndLimit  SystemSampleTime=-1  VariantActivationTime=update diagram  Latency=0  AutoFrameSizeCalculation=off
      link override Signal_Limit/_maxval: Value=KOUTP_StaFSya_flg_maxval
      link override Signal_Limit/_minval: Value=KOUTP_StaFSya_flg_minval
      link override Signal_Override/_ovrdflg: Value=KOUTP_StaFSya_flg_ovrdflg
      link override Signal_Override/_ovrdval: Value=KOUTP_StaFSya_flg_ovrdval
  VAPM_TCSActiveTimeOut_flg_Inproc : FVT_lib/outp/OverrideAndLimit  SystemSampleTime=-1  VariantActivationTime=update diagram  Latency=0  AutoFrameSizeCalculation=off
      link override Signal_Limit/_maxval: Value=KOUTP_TCSActiveTimeOut_flg_maxval
      link override Signal_Limit/_minval: Value=KOUTP_TCSActiveTimeOut_flg_minval
      link override Signal_Override/_ovrdflg: Value=KOUTP_TCSActiveTimeOut_flg_ovrdflg
      link override Signal_Override/_ovrdval: Value=KOUTP_TCSActiveTimeOut_flg_ovrdval
  VAPM_TCSActive_flg_Inproc : FVT_lib/outp/OverrideAndLimit  SystemSampleTime=-1  VariantActivationTime=update diagram  Latency=0  AutoFrameSizeCalculation=off
      link override Signal_Limit/_maxval: Value=KOUTP_TCSActive_flg_maxval
      link override Signal_Limit/_minval: Value=KOUTP_TCSActive_flg_minval
      link override Signal_Override/_ovrdflg: Value=KOUTP_TCSActive_flg_ovrdflg
      link override Signal_Override/_ovrdval: Value=KOUTP_TCSActive_flg_ovrdval
  VAPM_USSStaFCL_flg_Inproc : FVT_lib/outp/OverrideAndLimit  SystemSampleTime=-1  VariantActivationTime=update diagram  Latency=0  AutoFrameSizeCalculation=off
      link override Signal_Limit/_maxval: Value=KOUTP_USSStaFCL_flg_maxval
      link override Signal_Limit/_minval: Value=KOUTP_USSStaFCL_flg_minval
      link override Signal_Override/_ovrdflg: Value=KOUTP_USSStaFCL_flg_ovrdflg
      link override Signal_Override/_ovrdval: Value=KOUTP_USSStaFCL_flg_ovrdval
  VAPM_USSStaFCR_flg_Inproc : FVT_lib/outp/OverrideAndLimit  SystemSampleTime=-1  VariantActivationTime=update diagram  Latency=0  AutoFrameSizeCalculation=off
      link override Signal_Limit/_maxval: Value=KOUTP_USSStaFCR_flg_maxval
      link override Signal_Limit/_minval: Value=KOUTP_USSStaFCR_flg_minval
      link override Signal_Override/_ovrdflg: Value=KOUTP_USSStaFCR_flg_ovrdflg
      link override Signal_Override/_ovrdval: Value=KOUTP_USSStaFCR_flg_ovrdval
  VAPM_USSStaFLL_flg_Inproc : FVT_lib/outp/OverrideAndLimit  SystemSampleTime=-1  VariantActivationTime=update diagram  Latency=0  AutoFrameSizeCalculation=off
      link override Signal_Limit/_maxval: Value=KOUTP_USSStaFLL_flg_maxval
      link override Signal_Limit/_minval: Value=KOUTP_USSStaFLL_flg_minval
      link override Signal_Override/_ovrdflg: Value=KOUTP_USSStaFLL_flg_ovrdflg
      link override Signal_Override/_ovrdval: Value=KOUTP_USSStaFLL_flg_ovrdval
  VAPM_USSStaFLR_flg_Inproc : FVT_lib/outp/OverrideAndLimit  SystemSampleTime=-1  VariantActivationTime=update diagram  Latency=0  AutoFrameSizeCalculation=off
      link override Signal_Limit/_maxval: Value=KOUTP_USSStaFLR_flg_maxval
      link override Signal_Limit/_minval: Value=KOUTP_USSStaFLR_flg_minval
      link override Signal_Override/_ovrdflg: Value=KOUTP_USSStaFLR_flg_ovrdflg
      link override Signal_Override/_ovrdval: Value=KOUTP_USSStaFLR_flg_ovrdval
  VAPM_USSStaFML_flg_Inproc : FVT_lib/outp/OverrideAndLimit  SystemSampleTime=-1  VariantActivationTime=update diagram  Latency=0  AutoFrameSizeCalculation=off
      link override Signal_Limit/_maxval: Value=KOUTP_USSStaFML_flg_maxval
      link override Signal_Limit/_minval: Value=KOUTP_USSStaFML_flg_minval
      link override Signal_Override/_ovrdflg: Value=KOUTP_USSStaFML_flg_ovrdflg
      link override Signal_Override/_ovrdval: Value=KOUTP_USSStaFML_flg_ovrdval
  VAPM_USSStaFMR_flg_Inproc : FVT_lib/outp/OverrideAndLimit  SystemSampleTime=-1  VariantActivationTime=update diagram  Latency=0  AutoFrameSizeCalculation=off
      link override Signal_Limit/_maxval: Value=KOUTP_USSStaFMR_flg_maxval
      link override Signal_Limit/_minval: Value=KOUTP_USSStaFMR_flg_minval
      link override Signal_Override/_ovrdflg: Value=KOUTP_USSStaFMR_flg_ovrdflg
      link override Signal_Override/_ovrdval: Value=KOUTP_USSStaFMR_flg_ovrdval
  VAPM_USSStaRCL_flg_Inproc : FVT_lib/outp/OverrideAndLimit  SystemSampleTime=-1  VariantActivationTime=update diagram  Latency=0  AutoFrameSizeCalculation=off
      link override Signal_Limit/_maxval: Value=KOUTP_USSStaRCL_flg_maxval
      link override Signal_Limit/_minval: Value=KOUTP_USSStaRCL_flg_minval
      link override Signal_Override/_ovrdflg: Value=KOUTP_USSStaRCL_flg_ovrdflg
      link override Signal_Override/_ovrdval: Value=KOUTP_USSStaRCL_flg_ovrdval
  VAPM_USSStaRCR_flg_Inproc : FVT_lib/outp/OverrideAndLimit  SystemSampleTime=-1  VariantActivationTime=update diagram  Latency=0  AutoFrameSizeCalculation=off
      link override Signal_Limit/_maxval: Value=KOUTP_USSStaRCR_flg_maxval
      link override Signal_Limit/_minval: Value=KOUTP_USSStaRCR_flg_minval
      link override Signal_Override/_ovrdflg: Value=KOUTP_USSStaRCR_flg_ovrdflg
      link override Signal_Override/_ovrdval: Value=KOUTP_USSStaRCR_flg_ovrdval
  VAPM_USSStaRLL_flg_Inproc : FVT_lib/outp/OverrideAndLimit  SystemSampleTime=-1  VariantActivationTime=update diagram  Latency=0  AutoFrameSizeCalculation=off
      link override Signal_Limit/_maxval: Value=KOUTP_USSStaRLL_flg_maxval
      link override Signal_Limit/_minval: Value=KOUTP_USSStaRLL_flg_minval
      link override Signal_Override/_ovrdflg: Value=KOUTP_USSStaRLL_flg_ovrdflg
      link override Signal_Override/_ovrdval: Value=KOUTP_USSStaRLL_flg_ovrdval
  VAPM_USSStaRLR_flg_Inproc : FVT_lib/outp/OverrideAndLimit  SystemSampleTime=-1  VariantActivationTime=update diagram  Latency=0  AutoFrameSizeCalculation=off
      link override Signal_Limit/_maxval: Value=KOUTP_USSStaRLR_flg_maxval
      link override Signal_Limit/_minval: Value=KOUTP_USSStaRLR_flg_minval
      link override Signal_Override/_ovrdflg: Value=KOUTP_USSStaRLR_flg_ovrdflg
      link override Signal_Override/_ovrdval: Value=KOUTP_USSStaRLR_flg_ovrdval
  VAPM_USSStaRML_flg_Inproc : FVT_lib/outp/OverrideAndLimit  SystemSampleTime=-1  VariantActivationTime=update diagram  Latency=0  AutoFrameSizeCalculation=off
      link override Signal_Limit/_maxval: Value=KOUTP_USSStaRML_flg_maxval
      link override Signal_Limit/_minval: Value=KOUTP_USSStaRML_flg_minval
      link override Signal_Override/_ovrdflg: Value=KOUTP_USSStaRML_flg_ovrdflg
      link override Signal_Override/_ovrdval: Value=KOUTP_USSStaRML_flg_ovrdval
  VAPM_USSStaRMR_flg_Inproc : FVT_lib/outp/OverrideAndLimit  SystemSampleTime=-1  VariantActivationTime=update diagram  Latency=0  AutoFrameSizeCalculation=off
      link override Signal_Limit/_maxval: Value=KOUTP_USSStaRMR_flg_maxval
      link override Signal_Limit/_minval: Value=KOUTP_USSStaRMR_flg_minval
      link override Signal_Override/_ovrdflg: Value=KOUTP_USSStaRMR_flg_ovrdflg
      link override Signal_Override/_ovrdval: Value=KOUTP_USSStaRMR_flg_ovrdval
  VAPM_VehSpeedTimeOut_flg_Inproc : FVT_lib/outp/OverrideAndLimit  SystemSampleTime=-1  VariantActivationTime=update diagram  Latency=0  AutoFrameSizeCalculation=off
      link override Signal_Limit/_maxval: Value=KOUTP_VehSpeedTimeOut_flg_maxval
      link override Signal_Limit/_minval: Value=KOUTP_VehSpeedTimeOut_flg_minval
      link override Signal_Override/_ovrdflg: Value=KOUTP_VehSpeedTimeOut_flg_ovrdflg
      link override Signal_Override/_ovrdval: Value=KOUTP_VehSpeedTimeOut_flg_ovrdval
  VAPM_VehSpeed_kph_Inproc : FVT_lib/outp/OverrideAndLimit  SystemSampleTime=-1  VariantActivationTime=update diagram  Latency=0  AutoFrameSizeCalculation=off
      link override Signal_Limit/_maxval: Value=KOUTP_VehSpeed_kph_maxval
      link override Signal_Limit/_minval: Value=KOUTP_VehSpeed_kph_minval
      link override Signal_Override/_ovrdflg: Value=KOUTP_VehSpeed_kph_ovrdflg
      link override Signal_Override/_ovrdval: Value=KOUTP_VehSpeed_kph_ovrdval
  VAPM_YawRateTimeOut_flg_Inproc : FVT_lib/outp/OverrideAndLimit  SystemSampleTime=-1  VariantActivationTime=update diagram  Latency=0  AutoFrameSizeCalculation=off
      link override Signal_Limit/_maxval: Value=KOUTP_YawRateTimeOut_flg_maxval
      link override Signal_Limit/_minval: Value=KOUTP_YawRateTimeOut_flg_minval
      link override Signal_Override/_ovrdflg: Value=KOUTP_YawRateTimeOut_flg_ovrdflg
      link override Signal_Override/_ovrdval: Value=KOUTP_YawRateTimeOut_flg_ovrdval
  VAPM_YawRateVTimeOut_flg_Inproc : FVT_lib/outp/OverrideAndLimit  SystemSampleTime=-1  VariantActivationTime=update diagram  Latency=0  AutoFrameSizeCalculation=off
      link override Signal_Limit/_maxval: Value=KOUTP_YawRateVTimeOut_flg_maxval
      link override Signal_Limit/_minval: Value=KOUTP_YawRateVTimeOut_flg_minval
      link override Signal_Override/_ovrdflg: Value=KOUTP_YawRateVTimeOut_flg_ovrdflg
      link override Signal_Override/_ovrdval: Value=KOUTP_YawRateVTimeOut_flg_ovrdval
  VAPM_YawRateV_flg_Inproc : FVT_lib/outp/OverrideAndLimit  SystemSampleTime=-1  VariantActivationTime=update diagram  Latency=0  AutoFrameSizeCalculation=off
      link override Signal_Limit/_maxval: Value=KOUTP_YawRateV_flg_maxval
      link override Signal_Limit/_minval: Value=KOUTP_YawRateV_flg_minval
      link override Signal_Override/_ovrdflg: Value=KOUTP_YawRateV_flg_ovrdflg
      link override Signal_Override/_ovrdval: Value=KOUTP_YawRateV_flg_ovrdval
  VAPM_YawRate_degps_Inproc : FVT_lib/outp/OverrideAndLimit  SystemSampleTime=-1  VariantActivationTime=update diagram  Latency=0  AutoFrameSizeCalculation=off
      link override Signal_Limit/_maxval: Value=KOUTP_YawRate_degps_maxval
      link override Signal_Limit/_minval: Value=KOUTP_YawRate_degps_minval
      link override Signal_Override/_ovrdflg: Value=KOUTP_YawRate_degps_ovrdflg
      link override Signal_Override/_ovrdval: Value=KOUTP_YawRate_degps_ovrdval
  VBCM_APMDoorControlSta_flg_Inproc : FVT_lib/outp/OverrideAndLimit  SystemSampleTime=-1  VariantActivationTime=update diagram  Latency=0  AutoFrameSizeCalculation=off
      link override Signal_Limit/_maxval: Value=KOUTP_APMDoorControlSta_flg_maxval
      link override Signal_Limit/_minval: Value=KOUTP_APMDoorControlSta_flg_minval
      link override Signal_Override/_ovrdflg: Value=KOUTP_APMDoorControlSta_flg_ovrdflg
      link override Signal_Override/_ovrdval: Value=KOUTP_APMDoorControlSta_flg_ovrdval
  VBCM_APSOpenPTG_flg_Inproc : FVT_lib/outp/OverrideAndLimit  SystemSampleTime=-1  VariantActivationTime=update diagram  Latency=0  AutoFrameSizeCalculation=off
      link override Signal_Limit/_maxval: Value=KOUTP_APSOpenPTG_flg_maxval
      link override Signal_Limit/_minval: Value=KOUTP_APSOpenPTG_flg_minval
      link override Signal_Override/_ovrdflg: Value=KOUTP_APSOpenPTG_flg_ovrdflg
      link override Signal_Override/_ovrdval: Value=KOUTP_APSOpenPTG_flg_ovrdval
  VBCM_ATCtrl_enum_Inproc : FVT_lib/outp/OverrideAndLimit  SystemSampleTime=-1  VariantActivationTime=update diagram  Latency=0  AutoFrameSizeCalculation=off
      link override Signal_Limit/_maxval: Value=KOUTP_ATCtrl_enum_maxval
      link override Signal_Limit/_minval: Value=KOUTP_ATCtrl_enum_minval
      link override Signal_Override/_ovrdflg: Value=KOUTP_ATCtrl_enum_ovrdflg
      link override Signal_Override/_ovrdval: Value=KOUTP_ATCtrl_enum_ovrdval
  VBCM_AllDoorSW_flg_Inproc : FVT_lib/outp/OverrideAndLimit  SystemSampleTime=-1  VariantActivationTime=update diagram  Latency=0  AutoFrameSizeCalculation=off
      link override Signal_Limit/_maxval: Value=KOUTP_AllDoorSW_flg_maxval
      link override Signal_Limit/_minval: Value=KOUTP_AllDoorSW_flg_minval
      link override Signal_Override/_ovrdflg: Value=KOUTP_AllDoorSW_flg_ovrdflg
      link override Signal_Override/_ovrdval: Value=KOUTP_AllDoorSW_flg_ovrdval
  VBCM_AmbBrightSta_enum_Inproc : FVT_lib/outp/OverrideAndLimit  SystemSampleTime=-1  VariantActivationTime=update diagram  Latency=0  AutoFrameSizeCalculation=off
      link override Signal_Limit/_maxval: Value=KOUTP_AmbBrightSta_enum_maxval
      link override Signal_Limit/_minval: Value=KOUTP_AmbBrightSta_enum_minval
      link override Signal_Override/_ovrdflg: Value=KOUTP_AmbBrightSta_enum_ovrdflg
      link override Signal_Override/_ovrdval: Value=KOUTP_AmbBrightSta_enum_ovrdval
  VBCM_AmbBrightnessSta1_enum_Inproc : FVT_lib/outp/OverrideAndLimit  SystemSampleTime=-1  VariantActivationTime=update diagram  Latency=0  AutoFrameSizeCalculation=off
      link override Signal_Limit/_maxval: Value=KOUTP_AmbBrightnessSta1_enum_maxval
      link override Signal_Limit/_minval: Value=KOUTP_AmbBrightnessSta1_enum_minval
      link override Signal_Override/_ovrdflg: Value=KOUTP_AmbBrightnessSta1_enum_ovrdflg
      link override Signal_Override/_ovrdval: Value=KOUTP_AmbBrightnessSta1_enum_ovrdval
  VBCM_AmbBrightnessSta2_enum_Inproc : FVT_lib/outp/OverrideAndLimit  SystemSampleTime=-1  VariantActivationTime=update diagram  Latency=0  AutoFrameSizeCalculation=off
      link override Signal_Limit/_maxval: Value=KOUTP_AmbBrightnessSta2_enum_maxval
      link override Signal_Limit/_minval: Value=KOUTP_AmbBrightnessSta2_enum_minval
      link override Signal_Override/_ovrdflg: Value=KOUTP_AmbBrightnessSta2_enum_ovrdflg
      link override Signal_Override/_ovrdval: Value=KOUTP_AmbBrightnessSta2_enum_ovrdval
  VBCM_AmbBrightnessSta3_enum_Inproc : FVT_lib/outp/OverrideAndLimit  SystemSampleTime=-1  VariantActivationTime=update diagram  Latency=0  AutoFrameSizeCalculation=off
      link override Signal_Limit/_maxval: Value=KOUTP_AmbBrightnessSta3_enum_maxval
      link override Signal_Limit/_minval: Value=KOUTP_AmbBrightnessSta3_enum_minval
      link override Signal_Override/_ovrdflg: Value=KOUTP_AmbBrightnessSta3_enum_ovrdflg
      link override Signal_Override/_ovrdval: Value=KOUTP_AmbBrightnessSta3_enum_ovrdval
  VBCM_AmbBrightnessSta4_enum_Inproc : FVT_lib/outp/OverrideAndLimit  SystemSampleTime=-1  VariantActivationTime=update diagram  Latency=0  AutoFrameSizeCalculation=off
      link override Signal_Limit/_maxval: Value=KOUTP_AmbBrightnessSta4_enum_maxval
      link override Signal_Limit/_minval: Value=KOUTP_AmbBrightnessSta4_enum_minval
      link override Signal_Override/_ovrdflg: Value=KOUTP_AmbBrightnessSta4_enum_ovrdflg
      link override Signal_Override/_ovrdval: Value=KOUTP_AmbBrightnessSta4_enum_ovrdval
  VBCM_AmbBrightnessSta5_enum_Inproc : FVT_lib/outp/OverrideAndLimit  SystemSampleTime=-1  VariantActivationTime=update diagram  Latency=0  AutoFrameSizeCalculation=off
      link override Signal_Limit/_maxval: Value=KOUTP_AmbBrightnessSta5_enum_maxval
      link override Signal_Limit/_minval: Value=KOUTP_AmbBrightnessSta5_enum_minval
      link override Signal_Override/_ovrdflg: Value=KOUTP_AmbBrightnessSta5_enum_ovrdflg
      link override Signal_Override/_ovrdval: Value=KOUTP_AmbBrightnessSta5_enum_ovrdval
  VBCM_AmbBrightnessSta7_enum_Inproc : FVT_lib/outp/OverrideAndLimit  SystemSampleTime=-1  VariantActivationTime=update diagram  Latency=0  AutoFrameSizeCalculation=off
      link override Signal_Limit/_maxval: Value=KOUTP_AmbBrightnessSta7_enum_maxval
      link override Signal_Limit/_minval: Value=KOUTP_AmbBrightnessSta7_enum_minval
      link override Signal_Override/_ovrdflg: Value=KOUTP_AmbBrightnessSta7_enum_ovrdflg
      link override Signal_Override/_ovrdval: Value=KOUTP_AmbBrightnessSta7_enum_ovrdval
  VBCM_AmbColorSta1_enum_Inproc : FVT_lib/outp/OverrideAndLimit  SystemSampleTime=-1  VariantActivationTime=update diagram  Latency=0  AutoFrameSizeCalculation=off
      link override Signal_Limit/_maxval: Value=KOUTP_AmbColorSta1_enum_maxval
      link override Signal_Limit/_minval: Value=KOUTP_AmbColorSta1_enum_minval
      link override Signal_Override/_ovrdflg: Value=KOUTP_AmbColorSta1_enum_ovrdflg
      link override Signal_Override/_ovrdval: Value=KOUTP_AmbColorSta1_enum_ovrdval
  VBCM_AmbColorSta2_enum_Inproc : FVT_lib/outp/OverrideAndLimit  SystemSampleTime=-1  VariantActivationTime=update diagram  Latency=0  AutoFrameSizeCalculation=off
      link override Signal_Limit/_maxval: Value=KOUTP_AmbColorSta2_enum_maxval
      link override Signal_Limit/_minval: Value=KOUTP_AmbColorSta2_enum_minval
      link override Signal_Override/_ovrdflg: Value=KOUTP_AmbColorSta2_enum_ovrdflg
      link override Signal_Override/_ovrdval: Value=KOUTP_AmbColorSta2_enum_ovrdval
  VBCM_AmbColorSta3_enum_Inproc : FVT_lib/outp/OverrideAndLimit  SystemSampleTime=-1  VariantActivationTime=update diagram  Latency=0  AutoFrameSizeCalculation=off
      link override Signal_Limit/_maxval: Value=KOUTP_AmbColorSta3_enum_maxval
      link override Signal_Limit/_minval: Value=KOUTP_AmbColorSta3_enum_minval
      link override Signal_Override/_ovrdflg: Value=KOUTP_AmbColorSta3_enum_ovrdflg
      link override Signal_Override/_ovrdval: Value=KOUTP_AmbColorSta3_enum_ovrdval
  VBCM_AmbColorSta4_enum_Inproc : FVT_lib/outp/OverrideAndLimit  SystemSampleTime=-1  VariantActivationTime=update diagram  Latency=0  AutoFrameSizeCalculation=off
      link override Signal_Limit/_maxval: Value=KOUTP_AmbColorSta4_enum_maxval
      link override Signal_Limit/_minval: Value=KOUTP_AmbColorSta4_enum_minval
      link override Signal_Override/_ovrdflg: Value=KOUTP_AmbColorSta4_enum_ovrdflg
      link override Signal_Override/_ovrdval: Value=KOUTP_AmbColorSta4_enum_ovrdval
  VBCM_AmbColorSta5_enum_Inproc : FVT_lib/outp/OverrideAndLimit  SystemSampleTime=-1  VariantActivationTime=update diagram  Latency=0  AutoFrameSizeCalculation=off
      link override Signal_Limit/_maxval: Value=KOUTP_AmbColorSta5_enum_maxval
      link override Signal_Limit/_minval: Value=KOUTP_AmbColorSta5_enum_minval
      link override Signal_Override/_ovrdflg: Value=KOUTP_AmbColorSta5_enum_ovrdflg
      link override Signal_Override/_ovrdval: Value=KOUTP_AmbColorSta5_enum_ovrdval
  VBCM_AmbColorSta7_enum_Inproc : FVT_lib/outp/OverrideAndLimit  SystemSampleTime=-1  VariantActivationTime=update diagram  Latency=0  AutoFrameSizeCalculation=off
      link override Signal_Limit/_maxval: Value=KOUTP_AmbColorSta7_enum_maxval
      link override Signal_Limit/_minval: Value=KOUTP_AmbColorSta7_enum_minval
      link override Signal_Override/_ovrdflg: Value=KOUTP_AmbColorSta7_enum_ovrdflg
      link override Signal_Override/_ovrdval: Value=KOUTP_AmbColorSta7_enum_ovrdval
  VBCM_AmbColorSta_enum_Inproc : FVT_lib/outp/OverrideAndLimit  SystemSampleTime=-1  VariantActivationTime=update diagram  Latency=0  AutoFrameSizeCalculation=off
      link override Signal_Limit/_maxval: Value=KOUTP_AmbColorSta_enum_maxval
      link override Signal_Limit/_minval: Value=KOUTP_AmbColorSta_enum_minval
      link override Signal_Override/_ovrdflg: Value=KOUTP_AmbColorSta_enum_ovrdflg
      link override Signal_Override/_ovrdval: Value=KOUTP_AmbColorSta_enum_ovrdval
  VBCM_AmbDimENFlash_enum_Inproc : FVT_lib/outp/OverrideAndLimit  SystemSampleTime=-1  VariantActivationTime=update diagram  Latency=0  AutoFrameSizeCalculation=off
      link override Signal_Limit/_maxval: Value=KOUTP_AmbDimENFlash_enum_maxval
      link override Signal_Limit/_minval: Value=KOUTP_AmbDimENFlash_enum_minval
      link override Signal_Override/_ovrdflg: Value=KOUTP_AmbDimENFlash_enum_ovrdflg
      link override Signal_Override/_ovrdval: Value=KOUTP_AmbDimENFlash_enum_ovrdval
  VBCM_AmbDimEN_flg_Inproc : FVT_lib/outp/OverrideAndLimit  SystemSampleTime=-1  VariantActivationTime=update diagram  Latency=0  AutoFrameSizeCalculation=off
      link override Signal_Limit/_maxval: Value=KOUTP_AmbDimEN_flg_maxval
      link override Signal_Limit/_minval: Value=KOUTP_AmbDimEN_flg_minval
      link override Signal_Override/_ovrdflg: Value=KOUTP_AmbDimEN_flg_ovrdflg
      link override Signal_Override/_ovrdval: Value=KOUTP_AmbDimEN_flg_ovrdval
  VBCM_AmbFunENFlash_enum_Inproc : FVT_lib/outp/OverrideAndLimit  SystemSampleTime=-1  VariantActivationTime=update diagram  Latency=0  AutoFrameSizeCalculation=off
      link override Signal_Limit/_maxval: Value=KOUTP_AmbFunENFlash_enum_maxval
      link override Signal_Limit/_minval: Value=KOUTP_AmbFunENFlash_enum_minval
      link override Signal_Override/_ovrdflg: Value=KOUTP_AmbFunENFlash_enum_ovrdflg
      link override Signal_Override/_ovrdval: Value=KOUTP_AmbFunENFlash_enum_ovrdval
  VBCM_AmbFunEN_flg_Inproc : FVT_lib/outp/OverrideAndLimit  SystemSampleTime=-1  VariantActivationTime=update diagram  Latency=0  AutoFrameSizeCalculation=off
      link override Signal_Limit/_maxval: Value=KOUTP_AmbFunEN_flg_maxval
      link override Signal_Limit/_minval: Value=KOUTP_AmbFunEN_flg_minval
      link override Signal_Override/_ovrdflg: Value=KOUTP_AmbFunEN_flg_ovrdflg
      link override Signal_Override/_ovrdval: Value=KOUTP_AmbFunEN_flg_ovrdval
  VBCM_AmbLightBreath1_enum_Inproc : FVT_lib/outp/OverrideAndLimit  SystemSampleTime=-1  VariantActivationTime=update diagram  Latency=0  AutoFrameSizeCalculation=off
      link override Signal_Limit/_maxval: Value=KOUTP_AmbLightBreath1_enum_maxval
      link override Signal_Limit/_minval: Value=KOUTP_AmbLightBreath1_enum_minval
      link override Signal_Override/_ovrdflg: Value=KOUTP_AmbLightBreath1_enum_ovrdflg
      link override Signal_Override/_ovrdval: Value=KOUTP_AmbLightBreath1_enum_ovrdval
  VBCM_AmbLightBreath2_enum_Inproc : FVT_lib/outp/OverrideAndLimit  SystemSampleTime=-1  VariantActivationTime=update diagram  Latency=0  AutoFrameSizeCalculation=off
      link override Signal_Limit/_maxval: Value=KOUTP_AmbLightBreath2_enum_maxval
      link override Signal_Limit/_minval: Value=KOUTP_AmbLightBreath2_enum_minval
      link override Signal_Override/_ovrdflg: Value=KOUTP_AmbLightBreath2_enum_ovrdflg
      link override Signal_Override/_ovrdval: Value=KOUTP_AmbLightBreath2_enum_ovrdval
  VBCM_AmbLightBreath3_enum_Inproc : FVT_lib/outp/OverrideAndLimit  SystemSampleTime=-1  VariantActivationTime=update diagram  Latency=0  AutoFrameSizeCalculation=off
      link override Signal_Limit/_maxval: Value=KOUTP_AmbLightBreath3_enum_maxval
      link override Signal_Limit/_minval: Value=KOUTP_AmbLightBreath3_enum_minval
      link override Signal_Override/_ovrdflg: Value=KOUTP_AmbLightBreath3_enum_ovrdflg
      link override Signal_Override/_ovrdval: Value=KOUTP_AmbLightBreath3_enum_ovrdval
  VBCM_AmbLightBreath4_enum_Inproc : FVT_lib/outp/OverrideAndLimit  SystemSampleTime=-1  VariantActivationTime=update diagram  Latency=0  AutoFrameSizeCalculation=off
      link override Signal_Limit/_maxval: Value=KOUTP_AmbLightBreath4_enum_maxval
      link override Signal_Limit/_minval: Value=KOUTP_AmbLightBreath4_enum_minval
      link override Signal_Override/_ovrdflg: Value=KOUTP_AmbLightBreath4_enum_ovrdflg
      link override Signal_Override/_ovrdval: Value=KOUTP_AmbLightBreath4_enum_ovrdval
  VBCM_AmbLightBreath5_enum_Inproc : FVT_lib/outp/OverrideAndLimit  SystemSampleTime=-1  VariantActivationTime=update diagram  Latency=0  AutoFrameSizeCalculation=off
      link override Signal_Limit/_maxval: Value=KOUTP_AmbLightBreath5_enum_maxval
      link override Signal_Limit/_minval: Value=KOUTP_AmbLightBreath5_enum_minval
      link override Signal_Override/_ovrdflg: Value=KOUTP_AmbLightBreath5_enum_ovrdflg
      link override Signal_Override/_ovrdval: Value=KOUTP_AmbLightBreath5_enum_ovrdval
  VBCM_AmbLightBreath6_enum_Inproc : FVT_lib/outp/OverrideAndLimit  SystemSampleTime=-1  VariantActivationTime=update diagram  Latency=0  AutoFrameSizeCalculation=off
      link override Signal_Limit/_maxval: Value=KOUTP_AmbLightBreath6_enum_maxval
      link override Signal_Limit/_minval: Value=KOUTP_AmbLightBreath6_enum_minval
      link override Signal_Override/_ovrdflg: Value=KOUTP_AmbLightBreath6_enum_ovrdflg
      link override Signal_Override/_ovrdval: Value=KOUTP_AmbLightBreath6_enum_ovrdval
  VBCM_AmbLightBrightness1_enum_Inproc : FVT_lib/outp/OverrideAndLimit  SystemSampleTime=-1  VariantActivationTime=update diagram  Latency=0  AutoFrameSizeCalculation=off
      link override Signal_Limit/_maxval: Value=KOUTP_AmbLightBrightness1_enum_maxval
      link override Signal_Limit/_minval: Value=KOUTP_AmbLightBrightness1_enum_minval
      link override Signal_Override/_ovrdflg: Value=KOUTP_AmbLightBrightness1_enum_ovrdflg
      link override Signal_Override/_ovrdval: Value=KOUTP_AmbLightBrightness1_enum_ovrdval
  VBCM_AmbLightBrightness2_enum_Inproc : FVT_lib/outp/OverrideAndLimit  SystemSampleTime=-1  VariantActivationTime=update diagram  Latency=0  AutoFrameSizeCalculation=off
      link override Signal_Limit/_maxval: Value=KOUTP_AmbLightBrightness2_enum_maxval
      link override Signal_Limit/_minval: Value=KOUTP_AmbLightBrightness2_enum_minval
      link override Signal_Override/_ovrdflg: Value=KOUTP_AmbLightBrightness2_enum_ovrdflg
      link override Signal_Override/_ovrdval: Value=KOUTP_AmbLightBrightness2_enum_ovrdval
  VBCM_AmbLightBrightness3_enum_Inproc : FVT_lib/outp/OverrideAndLimit  SystemSampleTime=-1  VariantActivationTime=update diagram  Latency=0  AutoFrameSizeCalculation=off
      link override Signal_Limit/_maxval: Value=KOUTP_AmbLightBrightness3_enum_maxval
      link override Signal_Limit/_minval: Value=KOUTP_AmbLightBrightness3_enum_minval
      link override Signal_Override/_ovrdflg: Value=KOUTP_AmbLightBrightness3_enum_ovrdflg
      link override Signal_Override/_ovrdval: Value=KOUTP_AmbLightBrightness3_enum_ovrdval
  VBCM_AmbLightBrightness4_enum_Inproc : FVT_lib/outp/OverrideAndLimit  SystemSampleTime=-1  VariantActivationTime=update diagram  Latency=0  AutoFrameSizeCalculation=off
      link override Signal_Limit/_maxval: Value=KOUTP_AmbLightBrightness4_enum_maxval
      link override Signal_Limit/_minval: Value=KOUTP_AmbLightBrightness4_enum_minval
      link override Signal_Override/_ovrdflg: Value=KOUTP_AmbLightBrightness4_enum_ovrdflg
      link override Signal_Override/_ovrdval: Value=KOUTP_AmbLightBrightness4_enum_ovrdval
  VBCM_AmbLightBrightness5_enum_Inproc : FVT_lib/outp/OverrideAndLimit  SystemSampleTime=-1  VariantActivationTime=update diagram  Latency=0  AutoFrameSizeCalculation=off
      link override Signal_Limit/_maxval: Value=KOUTP_AmbLightBrightness5_enum_maxval
      link override Signal_Limit/_minval: Value=KOUTP_AmbLightBrightness5_enum_minval
      link override Signal_Override/_ovrdflg: Value=KOUTP_AmbLightBrightness5_enum_ovrdflg
      link override Signal_Override/_ovrdval: Value=KOUTP_AmbLightBrightness5_enum_ovrdval
  VBCM_AmbLightBrightness6_enum_Inproc : FVT_lib/outp/OverrideAndLimit  SystemSampleTime=-1  VariantActivationTime=update diagram  Latency=0  AutoFrameSizeCalculation=off
      link override Signal_Limit/_maxval: Value=KOUTP_AmbLightBrightness6_enum_maxval
      link override Signal_Limit/_minval: Value=KOUTP_AmbLightBrightness6_enum_minval
      link override Signal_Override/_ovrdflg: Value=KOUTP_AmbLightBrightness6_enum_ovrdflg
      link override Signal_Override/_ovrdval: Value=KOUTP_AmbLightBrightness6_enum_ovrdval
  VBCM_AmbLightColor1_enum_Inproc : FVT_lib/outp/OverrideAndLimit  SystemSampleTime=-1  VariantActivationTime=update diagram  Latency=0  AutoFrameSizeCalculation=off
      link override Signal_Limit/_maxval: Value=KOUTP_AmbLightColor1_enum_maxval
      link override Signal_Limit/_minval: Value=KOUTP_AmbLightColor1_enum_minval
      link override Signal_Override/_ovrdflg: Value=KOUTP_AmbLightColor1_enum_ovrdflg
      link override Signal_Override/_ovrdval: Value=KOUTP_AmbLightColor1_enum_ovrdval
  VBCM_AmbLightColor2_enum_Inproc : FVT_lib/outp/OverrideAndLimit  SystemSampleTime=-1  VariantActivationTime=update diagram  Latency=0  AutoFrameSizeCalculation=off
      link override Signal_Limit/_maxval: Value=KOUTP_AmbLightColor2_enum_maxval
      link override Signal_Limit/_minval: Value=KOUTP_AmbLightColor2_enum_minval
      link override Signal_Override/_ovrdflg: Value=KOUTP_AmbLightColor2_enum_ovrdflg
      link override Signal_Override/_ovrdval: Value=KOUTP_AmbLightColor2_enum_ovrdval
  VBCM_AmbLightColor3_enum_Inproc : FVT_lib/outp/OverrideAndLimit  SystemSampleTime=-1  VariantActivationTime=update diagram  Latency=0  AutoFrameSizeCalculation=off
      link override Signal_Limit/_maxval: Value=KOUTP_AmbLightColor3_enum_maxval
      link override Signal_Limit/_minval: Value=KOUTP_AmbLightColor3_enum_minval
      link override Signal_Override/_ovrdflg: Value=KOUTP_AmbLightColor3_enum_ovrdflg
      link override Signal_Override/_ovrdval: Value=KOUTP_AmbLightColor3_enum_ovrdval
  VBCM_AmbLightColor4_enum_Inproc : FVT_lib/outp/OverrideAndLimit  SystemSampleTime=-1  VariantActivationTime=update diagram  Latency=0  AutoFrameSizeCalculation=off
      link override Signal_Limit/_maxval: Value=KOUTP_AmbLightColor4_enum_maxval
      link override Signal_Limit/_minval: Value=KOUTP_AmbLightColor4_enum_minval
      link override Signal_Override/_ovrdflg: Value=KOUTP_AmbLightColor4_enum_ovrdflg
      link override Signal_Override/_ovrdval: Value=KOUTP_AmbLightColor4_enum_ovrdval
  VBCM_AmbLightColor5_enum_Inproc : FVT_lib/outp/OverrideAndLimit  SystemSampleTime=-1  VariantActivationTime=update diagram  Latency=0  AutoFrameSizeCalculation=off
      link override Signal_Limit/_maxval: Value=KOUTP_AmbLightColor5_enum_maxval
      link override Signal_Limit/_minval: Value=KOUTP_AmbLightColor5_enum_minval
      link override Signal_Override/_ovrdflg: Value=KOUTP_AmbLightColor5_enum_ovrdflg
      link override Signal_Override/_ovrdval: Value=KOUTP_AmbLightColor5_enum_ovrdval
  VBCM_AmbLightColor6_enum_Inproc : FVT_lib/outp/OverrideAndLimit  SystemSampleTime=-1  VariantActivationTime=update diagram  Latency=0  AutoFrameSizeCalculation=off
      link override Signal_Limit/_maxval: Value=KOUTP_AmbLightColor6_enum_maxval
      link override Signal_Limit/_minval: Value=KOUTP_AmbLightColor6_enum_minval
      link override Signal_Override/_ovrdflg: Value=KOUTP_AmbLightColor6_enum_ovrdflg
      link override Signal_Override/_ovrdval: Value=KOUTP_AmbLightColor6_enum_ovrdval
  VBCM_AmbLinkDriStaFlash_enum_Inproc : FVT_lib/outp/OverrideAndLimit  SystemSampleTime=-1  VariantActivationTime=update diagram  Latency=0  AutoFrameSizeCalculation=off
      link override Signal_Limit/_maxval: Value=KOUTP_AmbLinkDriStaFlash_enum_maxval
      link override Signal_Limit/_minval: Value=KOUTP_AmbLinkDriStaFlash_enum_minval
      link override Signal_Override/_ovrdflg: Value=KOUTP_AmbLinkDriStaFlash_enum_ovrdflg
      link override Signal_Override/_ovrdval: Value=KOUTP_AmbLinkDriStaFlash_enum_ovrdval
  VBCM_AmbLinkDriSta_flg_Inproc : FVT_lib/outp/OverrideAndLimit  SystemSampleTime=-1  VariantActivationTime=update diagram  Latency=0  AutoFrameSizeCalculation=off
      link override Signal_Limit/_maxval: Value=KOUTP_AmbLinkDriSta_flg_maxval
      link override Signal_Limit/_minval: Value=KOUTP_AmbLinkDriSta_flg_minval
      link override Signal_Override/_ovrdflg: Value=KOUTP_AmbLinkDriSta_flg_ovrdflg
      link override Signal_Override/_ovrdval: Value=KOUTP_AmbLinkDriSta_flg_ovrdval
  VBCM_AmbODAENFlash_enum_Inproc : FVT_lib/outp/OverrideAndLimit  SystemSampleTime=-1  VariantActivationTime=update diagram  Latency=0  AutoFrameSizeCalculation=off
      link override Signal_Limit/_maxval: Value=KOUTP_AmbODAENFlash_enum_maxval
      link override Signal_Limit/_minval: Value=KOUTP_AmbODAENFlash_enum_minval
      link override Signal_Override/_ovrdflg: Value=KOUTP_AmbODAENFlash_enum_ovrdflg
      link override Signal_Override/_ovrdval: Value=KOUTP_AmbODAENFlash_enum_ovrdval
  VBCM_AmbODAEN_flg_Inproc : FVT_lib/outp/OverrideAndLimit  SystemSampleTime=-1  VariantActivationTime=update diagram  Latency=0  AutoFrameSizeCalculation=off
      link override Signal_Limit/_maxval: Value=KOUTP_AmbODAEN_flg_maxval
      link override Signal_Limit/_minval: Value=KOUTP_AmbODAEN_flg_minval
      link override Signal_Override/_ovrdflg: Value=KOUTP_AmbODAEN_flg_ovrdflg
      link override Signal_Override/_ovrdval: Value=KOUTP_AmbODAEN_flg_ovrdval
  VBCM_AmbPwrWarnENFlash_enum_Inproc : FVT_lib/outp/OverrideAndLimit  SystemSampleTime=-1  VariantActivationTime=update diagram  Latency=0  AutoFrameSizeCalculation=off
      link override Signal_Limit/_maxval: Value=KOUTP_AmbPwrWarnENFlash_enum_maxval
      link override Signal_Limit/_minval: Value=KOUTP_AmbPwrWarnENFlash_enum_minval
      link override Signal_Override/_ovrdflg: Value=KOUTP_AmbPwrWarnENFlash_enum_ovrdflg
      link override Signal_Override/_ovrdval: Value=KOUTP_AmbPwrWarnENFlash_enum_ovrdval
  VBCM_AmbPwrWarnEN_flg_Inproc : FVT_lib/outp/OverrideAndLimit  SystemSampleTime=-1  VariantActivationTime=update diagram  Latency=0  AutoFrameSizeCalculation=off
      link override Signal_Limit/_maxval: Value=KOUTP_AmbPwrWarnEN_flg_maxval
      link override Signal_Limit/_minval: Value=KOUTP_AmbPwrWarnEN_flg_minval
      link override Signal_Override/_ovrdflg: Value=KOUTP_AmbPwrWarnEN_flg_ovrdflg
      link override Signal_Override/_ovrdval: Value=KOUTP_AmbPwrWarnEN_flg_ovrdval
  VBCM_AmbWelENFlash_enum_Inproc : FVT_lib/outp/OverrideAndLimit  SystemSampleTime=-1  VariantActivationTime=update diagram  Latency=0  AutoFrameSizeCalculation=off
      link override Signal_Limit/_maxval: Value=KOUTP_AmbWelENFlash_enum_maxval
      link override Signal_Limit/_minval: Value=KOUTP_AmbWelENFlash_enum_minval
      link override Signal_Override/_ovrdflg: Value=KOUTP_AmbWelENFlash_enum_ovrdflg
      link override Signal_Override/_ovrdval: Value=KOUTP_AmbWelENFlash_enum_ovrdval
  VBCM_AmbWelEN_flg_Inproc : FVT_lib/outp/OverrideAndLimit  SystemSampleTime=-1  VariantActivationTime=update diagram  Latency=0  AutoFrameSizeCalculation=off
      link override Signal_Limit/_maxval: Value=KOUTP_AmbWelEN_flg_maxval
      link override Signal_Limit/_minval: Value=KOUTP_AmbWelEN_flg_minval
      link override Signal_Override/_ovrdflg: Value=KOUTP_AmbWelEN_flg_ovrdflg
      link override Signal_Override/_ovrdval: Value=KOUTP_AmbWelEN_flg_ovrdval
  VBCM_AntitheftSeatFlod_flg_Inproc : FVT_lib/outp/OverrideAndLimit  SystemSampleTime=-1  VariantActivationTime=update diagram  Latency=0  AutoFrameSizeCalculation=off
      link override Signal_Limit/_maxval: Value=KOUTP_AntitheftSeatFlod_flg_maxval
      link override Signal_Limit/_minval: Value=KOUTP_AntitheftSeatFlod_flg_minval
      link override Signal_Override/_ovrdflg: Value=KOUTP_AntitheftSeatFlod_flg_ovrdflg
      link override Signal_Override/_ovrdval: Value=KOUTP_AntitheftSeatFlod_flg_ovrdval
  VBCM_AntitheftSta_enum_Inproc : FVT_lib/outp/OverrideAndLimit  SystemSampleTime=-1  VariantActivationTime=update diagram  Latency=0  AutoFrameSizeCalculation=off
      link override Signal_Limit/_maxval: Value=KOUTP_AntitheftSta_enum_maxval
      link override Signal_Limit/_minval: Value=KOUTP_AntitheftSta_enum_minval
      link override Signal_Override/_ovrdflg: Value=KOUTP_AntitheftSta_enum_ovrdflg
      link override Signal_Override/_ovrdval: Value=KOUTP_AntitheftSta_enum_ovrdval
  VBCM_BCMBuzzerReq_flg_Inproc : FVT_lib/outp/OverrideAndLimit  SystemSampleTime=-1  VariantActivationTime=update diagram  Latency=0  AutoFrameSizeCalculation=off
      link override Signal_Limit/_maxval: Value=KOUTP_BCMBuzzerReq_flg_maxval
      link override Signal_Limit/_minval: Value=KOUTP_BCMBuzzerReq_flg_minval
      link override Signal_Override/_ovrdflg: Value=KOUTP_BCMBuzzerReq_flg_ovrdflg
      link override Signal_Override/_ovrdval: Value=KOUTP_BCMBuzzerReq_flg_ovrdval
  VBCM_BCMDoorLockSta_flg_Inproc : FVT_lib/outp/OverrideAndLimit  SystemSampleTime=-1  VariantActivationTime=update diagram  Latency=0  AutoFrameSizeCalculation=off
      link override Signal_Limit/_maxval: Value=KOUTP_BCMDoorLockSta_flg_maxval
      link override Signal_Limit/_minval: Value=KOUTP_BCMDoorLockSta_flg_minval
      link override Signal_Override/_ovrdflg: Value=KOUTP_BCMDoorLockSta_flg_ovrdflg
      link override Signal_Override/_ovrdval: Value=KOUTP_BCMDoorLockSta_flg_ovrdval
  VBCM_BrakeLamp_flg_Inproc : FVT_lib/outp/OverrideAndLimit  SystemSampleTime=-1  VariantActivationTime=update diagram  Latency=0  AutoFrameSizeCalculation=off
      link override Signal_Limit/_maxval: Value=KOUTP_BrakeLamp_flg_maxval
      link override Signal_Limit/_minval: Value=KOUTP_BrakeLamp_flg_minval
      link override Signal_Override/_ovrdflg: Value=KOUTP_BrakeLamp_flg_ovrdflg
      link override Signal_Override/_ovrdval: Value=KOUTP_BrakeLamp_flg_ovrdval
  VBCM_CTDCtrl_enum_Inproc : FVT_lib/outp/OverrideAndLimit  SystemSampleTime=-1  VariantActivationTime=update diagram  Latency=0  AutoFrameSizeCalculation=off
      link override Signal_Limit/_maxval: Value=KOUTP_CTDCtrl_enum_maxval
      link override Signal_Limit/_minval: Value=KOUTP_CTDCtrl_enum_minval
      link override Signal_Override/_ovrdflg: Value=KOUTP_CTDCtrl_enum_ovrdflg
      link override Signal_Override/_ovrdval: Value=KOUTP_CTDCtrl_enum_ovrdval
  VBCM_CTDLockSW_flg_Inproc : FVT_lib/outp/OverrideAndLimit  SystemSampleTime=-1  VariantActivationTime=update diagram  Latency=0  AutoFrameSizeCalculation=off
      link override Signal_Limit/_maxval: Value=KOUTP_CTDLockSW_flg_maxval
      link override Signal_Limit/_minval: Value=KOUTP_CTDLockSW_flg_minval
      link override Signal_Override/_ovrdflg: Value=KOUTP_CTDLockSW_flg_ovrdflg
      link override Signal_Override/_ovrdval: Value=KOUTP_CTDLockSW_flg_ovrdval
